simulink model "SUB_ExpIOControl"  (R2018b)
(part 5 of 6)

  out_OUT_ACAN.BSG_EXPA.OUT_12 : KIBES_Signal/KIBES_Signal  MBDS_LibraryBlock=on  DatabaseKey=932  SignalName=OUT_ACAN.BSG_EXPA.OUT_12  SymbolName=OUT_ACAN_BSG_EXPA_OUT_12_000932  DataType=boolean  Init=0  Slope=1  Bias=0  DataSize=1  fpDataType=boolean  BlockIOType=Outport  DeviceType=0
  out_OUT_ACAN.BSG_EXPA.OUT_12_TD_START : KIBES_Signal/KIBES_Signal  MBDS_LibraryBlock=on  DatabaseKey=928  SignalName=OUT_ACAN.BSG_EXPA.OUT_12_TD_START  SymbolName=OUT_ACAN_BSG_EXPA_OUT_12_TD_START_000928  DataType=boolean  Init=0  Slope=1  Bias=0  DataSize=1  fpDataType=boolean  BlockIOType=Outport  DeviceType=0
  out_OUT_ACAN.BSG_EXPA.OUT_13 : KIBES_Signal/KIBES_Signal  MBDS_LibraryBlock=on  DatabaseKey=911  SignalName=OUT_ACAN.BSG_EXPA.OUT_13  SymbolName=OUT_ACAN_BSG_EXPA_OUT_13_000911  DataType=boolean  Init=0  Slope=1  Bias=0  DataSize=1  fpDataType=boolean  BlockIOType=Outport  DeviceType=0
  out_OUT_ACAN.BSG_EXPA.OUT_14 : KIBES_Signal/KIBES_Signal  MBDS_LibraryBlock=on  DatabaseKey=964  SignalName=OUT_ACAN.BSG_EXPA.OUT_14  SymbolName=OUT_ACAN_BSG_EXPA_OUT_14_000964  DataType=boolean  Init=0  Slope=1  Bias=0  DataSize=1  fpDataType=boolean  BlockIOType=Outport  DeviceType=0
  out_OUT_ACAN.BSG_EXPA.OUT_15 : KIBES_Signal/KIBES_Signal  MBDS_LibraryBlock=on  DatabaseKey=924  SignalName=OUT_ACAN.BSG_EXPA.OUT_15  SymbolName=OUT_ACAN_BSG_EXPA_OUT_15_000924  DataType=boolean  Init=0  Slope=1  Bias=0  DataSize=1  fpDataType=boolean  BlockIOType=Outport  DeviceType=0
  out_OUT_ACAN.BSG_EXPA.OUT_16 : KIBES_Signal/KIBES_Signal  MBDS_LibraryBlock=on  DatabaseKey=921  SignalName=OUT_ACAN.BSG_EXPA.OUT_16  SymbolName=OUT_ACAN_BSG_EXPA_OUT_16_000921  DataType=boolean  Init=0  Slope=1  Bias=0  DataSize=1  fpDataType=boolean  BlockIOType=Outport  DeviceType=0
  out_OUT_ACAN.BSG_EXPA.OUT_17 : KIBES_Signal/KIBES_Signal  MBDS_LibraryBlock=on  DatabaseKey=946  SignalName=OUT_ACAN.BSG_EXPA.OUT_17  SymbolName=OUT_ACAN_BSG_EXPA_OUT_17_000946  DataType=boolean  Init=0  Slope=1  Bias=0  DataSize=1  fpDataType=boolean  BlockIOType=Outport  DeviceType=0
  out_OUT_ACAN.BSG_EXPA.OUT_18 : KIBES_Signal/KIBES_Signal  MBDS_LibraryBlock=on  DatabaseKey=943  SignalName=OUT_ACAN.BSG_EXPA.OUT_18  SymbolName=OUT_ACAN_BSG_EXPA_OUT_18_000943  DataType=boolean  Init=0  Slope=1  Bias=0  DataSize=1  fpDataType=boolean  BlockIOType=Outport  DeviceType=0
  out_OUT_ACAN.BSG_EXPA.OUT_19 : KIBES_Signal/KIBES_Signal  MBDS_LibraryBlock=on  DatabaseKey=930  SignalName=OUT_ACAN.BSG_EXPA.OUT_19  SymbolName=OUT_ACAN_BSG_EXPA_OUT_19_000930  DataType=boolean  Init=0  Slope=1  Bias=0  DataSize=1  fpDataType=boolean  BlockIOType=Outport  DeviceType=0
  out_OUT_ACAN.BSG_EXPA.OUT_20 : KIBES_Signal/KIBES_Signal  MBDS_LibraryBlock=on  DatabaseKey=949  SignalName=OUT_ACAN.BSG_EXPA.OUT_20  SymbolName=OUT_ACAN_BSG_EXPA_OUT_20_000949  DataType=boolean  Init=0  Slope=1  Bias=0  DataSize=1  fpDataType=boolean  BlockIOType=Outport  DeviceType=0
  out_OUT_ACAN.BSG_EXPA.OUT_21 : KIBES_Signal/KIBES_Signal  MBDS_LibraryBlock=on  DatabaseKey=954  SignalName=OUT_ACAN.BSG_EXPA.OUT_21  SymbolName=OUT_ACAN_BSG_EXPA_OUT_21_000954  DataType=boolean  Init=0  Slope=1  Bias=0  DataSize=1  fpDataType=boolean  BlockIOType=Outport  DeviceType=0
  out_OUT_ACAN.BSG_EXPA.OUT_21_TD_START : KIBES_Signal/KIBES_Signal  MBDS_LibraryBlock=on  DatabaseKey=971  SignalName=OUT_ACAN.BSG_EXPA.OUT_21_TD_START  SymbolName=OUT_ACAN_BSG_EXPA_OUT_21_TD_START_000971  DataType=boolean  Init=0  Slope=1  Bias=0  DataSize=1  fpDataType=boolean  BlockIOType=Outport  DeviceType=0
  out_OUT_ACAN.BSG_EXPA.OUT_22 : KIBES_Signal/KIBES_Signal  MBDS_LibraryBlock=on  DatabaseKey=952  SignalName=OUT_ACAN.BSG_EXPA.OUT_22  SymbolName=OUT_ACAN_BSG_EXPA_OUT_22_000952  DataType=boolean  Init=0  Slope=1  Bias=0  DataSize=1  fpDataType=boolean  BlockIOType=Outport  DeviceType=0
  out_OUT_ACAN.BSG_EXPA.OUT_23 : KIBES_Signal/KIBES_Signal  MBDS_LibraryBlock=on  DatabaseKey=970  SignalName=OUT_ACAN.BSG_EXPA.OUT_23  SymbolName=OUT_ACAN_BSG_EXPA_OUT_23_000970  DataType=boolean  Init=0  Slope=1  Bias=0  DataSize=1  fpDataType=boolean  BlockIOType=Outport  DeviceType=0
  out_OUT_ACAN.BSG_EXPA.OUT_24 : KIBES_Signal/KIBES_Signal  MBDS_LibraryBlock=on  DatabaseKey=927  SignalName=OUT_ACAN.BSG_EXPA.OUT_24  SymbolName=OUT_ACAN_BSG_EXPA_OUT_24_000927  DataType=boolean  Init=0  Slope=1  Bias=0  DataSize=1  fpDataType=boolean  BlockIOType=Outport  DeviceType=0
  out_OUT_ACAN.BSG_EXPA.OUT_25 : KIBES_Signal/KIBES_Signal  MBDS_LibraryBlock=on  DatabaseKey=953  SignalName=OUT_ACAN.BSG_EXPA.OUT_25  SymbolName=OUT_ACAN_BSG_EXPA_OUT_25_000953  DataType=boolean  Init=0  Slope=1  Bias=0  DataSize=1  fpDataType=boolean  BlockIOType=Outport  DeviceType=0
  out_OUT_ACAN.BSG_EXPA.OUT_26 : KIBES_Signal/KIBES_Signal  MBDS_LibraryBlock=on  DatabaseKey=913  SignalName=OUT_ACAN.BSG_EXPA.OUT_26  SymbolName=OUT_ACAN_BSG_EXPA_OUT_26_000913  DataType=boolean  Init=0  Slope=1  Bias=0  DataSize=1  fpDataType=boolean  BlockIOType=Outport  DeviceType=0
  out_OUT_ACAN.BSG_EXPA.OUT_27 : KIBES_Signal/KIBES_Signal  MBDS_LibraryBlock=on  DatabaseKey=919  SignalName=OUT_ACAN.BSG_EXPA.OUT_27  SymbolName=OUT_ACAN_BSG_EXPA_OUT_27_000919  DataType=boolean  Init=0  Slope=1  Bias=0  DataSize=1  fpDataType=boolean  BlockIOType=Outport  DeviceType=0
  out_OUT_ACAN.BSG_EXPA.OUT_28 : KIBES_Signal/KIBES_Signal  MBDS_LibraryBlock=on  DatabaseKey=916  SignalName=OUT_ACAN.BSG_EXPA.OUT_28  SymbolName=OUT_ACAN_BSG_EXPA_OUT_28_000916  DataType=boolean  Init=0  Slope=1  Bias=0  DataSize=1  fpDataType=boolean  BlockIOType=Outport  DeviceType=0
  out_OUT_ACAN.BSG_EXPA.OUT_29_HB : KIBES_Signal/KIBES_Signal  MBDS_LibraryBlock=on  DatabaseKey=2301  SignalName=OUT_ACAN.BSG_EXPA.OUT_29_HB  SymbolName=OUT_ACAN_BSG_EXPA_OUT_29_HB_002301  DataType=int8  Init=0  Slope=1  Bias=0  DataSize=1  fpDataType=int8  BlockIOType=Outport  DeviceType=0
  out_OUT_ACAN.BSG_EXPA.OUT_30_HB : KIBES_Signal/KIBES_Signal  MBDS_LibraryBlock=on  DatabaseKey=2303  SignalName=OUT_ACAN.BSG_EXPA.OUT_30_HB  SymbolName=OUT_ACAN_BSG_EXPA_OUT_30_HB_002303  DataType=int8  Init=0  Slope=1  Bias=0  DataSize=1  fpDataType=int8  BlockIOType=Outport  DeviceType=0
  out_OUT_ACAN.BSG_EXPA.OUT_31_HB : KIBES_Signal/KIBES_Signal  MBDS_LibraryBlock=on  DatabaseKey=2305  SignalName=OUT_ACAN.BSG_EXPA.OUT_31_HB  SymbolName=OUT_ACAN_BSG_EXPA_OUT_31_HB_002305  DataType=int8  Init=0  Slope=1  Bias=0  DataSize=1  fpDataType=int8  BlockIOType=Outport  DeviceType=0
  out_OUT_ACAN.BSG_EXPA.OUT_32_HB : KIBES_Signal/KIBES_Signal  MBDS_LibraryBlock=on  DatabaseKey=2307  SignalName=OUT_ACAN.BSG_EXPA.OUT_32_HB  SymbolName=OUT_ACAN_BSG_EXPA_OUT_32_HB_002307  DataType=int8  Init=0  Slope=1  Bias=0  DataSize=1  fpDataType=int8  BlockIOType=Outport  DeviceType=0
  out_OUT_ACAN.BSG_EXPA.OUT_33_HB : KIBES_Signal/KIBES_Signal  MBDS_LibraryBlock=on  DatabaseKey=2309  SignalName=OUT_ACAN.BSG_EXPA.OUT_33_HB  SymbolName=OUT_ACAN_BSG_EXPA_OUT_33_HB_002309  DataType=int8  Init=0  Slope=1  Bias=0  DataSize=1  fpDataType=int8  BlockIOType=Outport  DeviceType=0
  out_OUT_ACAN.BSG_EXPA.OUT_34_HB : KIBES_Signal/KIBES_Signal  MBDS_LibraryBlock=on  DatabaseKey=2311  SignalName=OUT_ACAN.BSG_EXPA.OUT_34_HB  SymbolName=OUT_ACAN_BSG_EXPA_OUT_34_HB_002311  DataType=int8  Init=0  Slope=1  Bias=0  DataSize=1  fpDataType=int8  BlockIOType=Outport  DeviceType=0
  out_OUT_ACAN.BSG_EXPA.OUT_OLD_01 : KIBES_Signal/KIBES_Signal  MBDS_LibraryBlock=on  DatabaseKey=959  SignalName=OUT_ACAN.BSG_EXPA.OUT_OLD_01  SymbolName=OUT_ACAN_BSG_EXPA_OUT_OLD_01_000959  DataType=boolean  Init=0  Slope=1  Bias=0  DataSize=1  fpDataType=boolean  BlockIOType=Outport  DeviceType=0
  out_OUT_ACAN.BSG_EXPA.OUT_OLD_02 : KIBES_Signal/KIBES_Signal  MBDS_LibraryBlock=on  DatabaseKey=937  SignalName=OUT_ACAN.BSG_EXPA.OUT_OLD_02  SymbolName=OUT_ACAN_BSG_EXPA_OUT_OLD_02_000937  DataType=boolean  Init=0  Slope=1  Bias=0  DataSize=1  fpDataType=boolean  BlockIOType=Outport  DeviceType=0
  out_OUT_ACAN.BSG_EXPA.OUT_OLD_03 : KIBES_Signal/KIBES_Signal  MBDS_LibraryBlock=on  DatabaseKey=895  SignalName=OUT_ACAN.BSG_EXPA.OUT_OLD_03  SymbolName=OUT_ACAN_BSG_EXPA_OUT_OLD_03_000895  DataType=boolean  Init=0  Slope=1  Bias=0  DataSize=1  fpDataType=boolean  BlockIOType=Outport  DeviceType=0
  out_OUT_ACAN.BSG_EXPA.OUT_OLD_04 : KIBES_Signal/KIBES_Signal  MBDS_LibraryBlock=on  DatabaseKey=896  SignalName=OUT_ACAN.BSG_EXPA.OUT_OLD_04  SymbolName=OUT_ACAN_BSG_EXPA_OUT_OLD_04_000896  DataType=boolean  Init=0  Slope=1  Bias=0  DataSize=1  fpDataType=boolean  BlockIOType=Outport  DeviceType=0
  out_OUT_FMSCAN.Rx_Ctrl.Out_Ctrl.MessageEnable : KIBES_Signal/KIBES_Signal  MBDS_LibraryBlock=on  DatabaseKey=2679  SignalName=OUT_FMSCAN.Rx_Ctrl.Out_Ctrl.MessageEnable  SymbolName=OUT_FMSCAN_Rx_Ctrl_Out_Ctrl_MessageEnable_002679  DataType=boolean  Init=0  Slope=1  Bias=0  DataSize=1  fpDataType=boolean  BlockIOType=Outport  DeviceType=0
  out_OUT_FMSCAN.Rx_Ctrl.Out_HB_Ctrl.MessageEnable : KIBES_Signal/KIBES_Signal  MBDS_LibraryBlock=on  DatabaseKey=2681  SignalName=OUT_FMSCAN.Rx_Ctrl.Out_HB_Ctrl.MessageEnable  SymbolName=OUT_FMSCAN_Rx_Ctrl_Out_HB_Ctrl_MessageEnable_002681  DataType=boolean  Init=0  Slope=1  Bias=0  DataSize=1  fpDataType=boolean  BlockIOType=Outport  DeviceType=0
  out_OUT_FMSCAN.Rx_Ctrl.Out_Mirror_HB_Ctrl.MessageEnable : KIBES_Signal/KIBES_Signal  MBDS_LibraryBlock=on  DatabaseKey=2683  SignalName=OUT_FMSCAN.Rx_Ctrl.Out_Mirror_HB_Ctrl.MessageEnable  SymbolName=OUT_FMSCAN_Rx_Ctrl_Out_Mirror_HB_Ctrl_MessageEnable_002683  DataType=boolean  Init=0  Slope=1  Bias=0  DataSize=1  fpDataType=boolean  BlockIOType=Outport  DeviceType=0
  out_OUT_FMSCAN.Tx_Out.Out_01_Sts.MessageEnable : KIBES_Signal/KIBES_Signal  MBDS_LibraryBlock=on  DatabaseKey=2542  SignalName=OUT_FMSCAN.Tx_Out.Out_01_Sts.MessageEnable  SymbolName=OUT_FMSCAN_Tx_Out_Out_01_Sts_MessageEnable_002542  DataType=boolean  Init=0  Slope=1  Bias=0  DataSize=1  fpDataType=boolean  BlockIOType=Outport  DeviceType=0
  out_OUT_FMSCAN.Tx_Out.Out_01_Sts.Out_DIAG : KIBES_Signal/KIBES_Signal  MBDS_LibraryBlock=on  DatabaseKey=2432  SignalName=OUT_FMSCAN.Tx_Out.Out_01_Sts.Out_DIAG  SymbolName=OUT_FMSCAN_Tx_Out_Out_01_Sts_Out_DIAG_002432  DataType=uint16  Init=0  Slope=1  Bias=0  DataSize=1  fpDataType=uint16  BlockIOType=Outport  DeviceType=0
  out_OUT_FMSCAN.Tx_Out.Out_01_Sts.Out_SENSE : KIBES_Signal/KIBES_Signal  MBDS_LibraryBlock=on  DatabaseKey=2433  SignalName=OUT_FMSCAN.Tx_Out.Out_01_Sts.Out_SENSE  SymbolName=OUT_FMSCAN_Tx_Out_Out_01_Sts_Out_SENSE_002433  DataType=uint16  Init=0  Slope=1  Bias=0  DataSize=1  fpDataType=uint16  BlockIOType=Outport  DeviceType=0
  out_OUT_FMSCAN.Tx_Out.Out_01_Sts.Out_STATUS : KIBES_Signal/KIBES_Signal  MBDS_LibraryBlock=on  DatabaseKey=2434  SignalName=OUT_FMSCAN.Tx_Out.Out_01_Sts.Out_STATUS  SymbolName=OUT_FMSCAN_Tx_Out_Out_01_Sts_Out_STATUS_002434  DataType=uint8  Init=0  Slope=1  Bias=0  DataSize=1  fpDataType=uint8  BlockIOType=Outport  DeviceType=0
  out_OUT_FMSCAN.Tx_Out.Out_02_Sts.MessageEnable : KIBES_Signal/KIBES_Signal  MBDS_LibraryBlock=on  DatabaseKey=2543  SignalName=OUT_FMSCAN.Tx_Out.Out_02_Sts.MessageEnable  SymbolName=OUT_FMSCAN_Tx_Out_Out_02_Sts_MessageEnable_002543  DataType=boolean  Init=0  Slope=1  Bias=0  DataSize=1  fpDataType=boolean  BlockIOType=Outport  DeviceType=0
  out_OUT_FMSCAN.Tx_Out.Out_02_Sts.Out_DIAG : KIBES_Signal/KIBES_Signal  MBDS_LibraryBlock=on  DatabaseKey=2435  SignalName=OUT_FMSCAN.Tx_Out.Out_02_Sts.Out_DIAG  SymbolName=OUT_FMSCAN_Tx_Out_Out_02_Sts_Out_DIAG_002435  DataType=uint16  Init=0  Slope=1  Bias=0  DataSize=1  fpDataType=uint16  BlockIOType=Outport  DeviceType=0
  out_OUT_FMSCAN.Tx_Out.Out_02_Sts.Out_SENSE : KIBES_Signal/KIBES_Signal  MBDS_LibraryBlock=on  DatabaseKey=2436  SignalName=OUT_FMSCAN.Tx_Out.Out_02_Sts.Out_SENSE  SymbolName=OUT_FMSCAN_Tx_Out_Out_02_Sts_Out_SENSE_002436  DataType=uint16  Init=0  Slope=1  Bias=0  DataSize=1  fpDataType=uint16  BlockIOType=Outport  DeviceType=0
  out_OUT_FMSCAN.Tx_Out.Out_02_Sts.Out_STATUS : KIBES_Signal/KIBES_Signal  MBDS_LibraryBlock=on  DatabaseKey=2437  SignalName=OUT_FMSCAN.Tx_Out.Out_02_Sts.Out_STATUS  SymbolName=OUT_FMSCAN_Tx_Out_Out_02_Sts_Out_STATUS_002437  DataType=uint8  Init=0  Slope=1  Bias=0  DataSize=1  fpDataType=uint8  BlockIOType=Outport  DeviceType=0
  out_OUT_FMSCAN.Tx_Out.Out_03_Sts.MessageEnable : KIBES_Signal/KIBES_Signal  MBDS_LibraryBlock=on  DatabaseKey=2544  SignalName=OUT_FMSCAN.Tx_Out.Out_03_Sts.MessageEnable  SymbolName=OUT_FMSCAN_Tx_Out_Out_03_Sts_MessageEnable_002544  DataType=boolean  Init=0  Slope=1  Bias=0  DataSize=1  fpDataType=boolean  BlockIOType=Outport  DeviceType=0
  out_OUT_FMSCAN.Tx_Out.Out_03_Sts.Out_DIAG : KIBES_Signal/KIBES_Signal  MBDS_LibraryBlock=on  DatabaseKey=2438  SignalName=OUT_FMSCAN.Tx_Out.Out_03_Sts.Out_DIAG  SymbolName=OUT_FMSCAN_Tx_Out_Out_03_Sts_Out_DIAG_002438  DataType=uint16  Init=0  Slope=1  Bias=0  DataSize=1  fpDataType=uint16  BlockIOType=Outport  DeviceType=0
  out_OUT_FMSCAN.Tx_Out.Out_03_Sts.Out_SENSE : KIBES_Signal/KIBES_Signal  MBDS_LibraryBlock=on  DatabaseKey=2439  SignalName=OUT_FMSCAN.Tx_Out.Out_03_Sts.Out_SENSE  SymbolName=OUT_FMSCAN_Tx_Out_Out_03_Sts_Out_SENSE_002439  DataType=uint16  Init=0  Slope=1  Bias=0  DataSize=1  fpDataType=uint16  BlockIOType=Outport  DeviceType=0
  out_OUT_FMSCAN.Tx_Out.Out_03_Sts.Out_STATUS : KIBES_Signal/KIBES_Signal  MBDS_LibraryBlock=on  DatabaseKey=2440  SignalName=OUT_FMSCAN.Tx_Out.Out_03_Sts.Out_STATUS  SymbolName=OUT_FMSCAN_Tx_Out_Out_03_Sts_Out_STATUS_002440  DataType=uint8  Init=0  Slope=1  Bias=0  DataSize=1  fpDataType=uint8  BlockIOType=Outport  DeviceType=0
  out_OUT_FMSCAN.Tx_Out.Out_04_Sts.MessageEnable : KIBES_Signal/KIBES_Signal  MBDS_LibraryBlock=on  DatabaseKey=2545  SignalName=OUT_FMSCAN.Tx_Out.Out_04_Sts.MessageEnable  SymbolName=OUT_FMSCAN_Tx_Out_Out_04_Sts_MessageEnable_002545  DataType=boolean  Init=0  Slope=1  Bias=0  DataSize=1  fpDataType=boolean  BlockIOType=Outport  DeviceType=0
  out_OUT_FMSCAN.Tx_Out.Out_04_Sts.Out_DIAG : KIBES_Signal/KIBES_Signal  MBDS_LibraryBlock=on  DatabaseKey=2441  SignalName=OUT_FMSCAN.Tx_Out.Out_04_Sts.Out_DIAG  SymbolName=OUT_FMSCAN_Tx_Out_Out_04_Sts_Out_DIAG_002441  DataType=uint16  Init=0  Slope=1  Bias=0  DataSize=1  fpDataType=uint16  BlockIOType=Outport  DeviceType=0
  out_OUT_FMSCAN.Tx_Out.Out_04_Sts.Out_SENSE : KIBES_Signal/KIBES_Signal  MBDS_LibraryBlock=on  DatabaseKey=2442  SignalName=OUT_FMSCAN.Tx_Out.Out_04_Sts.Out_SENSE  SymbolName=OUT_FMSCAN_Tx_Out_Out_04_Sts_Out_SENSE_002442  DataType=uint16  Init=0  Slope=1  Bias=0  DataSize=1  fpDataType=uint16  BlockIOType=Outport  DeviceType=0
  out_OUT_FMSCAN.Tx_Out.Out_04_Sts.Out_STATUS : KIBES_Signal/KIBES_Signal  MBDS_LibraryBlock=on  DatabaseKey=2443  SignalName=OUT_FMSCAN.Tx_Out.Out_04_Sts.Out_STATUS  SymbolName=OUT_FMSCAN_Tx_Out_Out_04_Sts_Out_STATUS_002443  DataType=uint8  Init=0  Slope=1  Bias=0  DataSize=1  fpDataType=uint8  BlockIOType=Outport  DeviceType=0
  out_OUT_FMSCAN.Tx_Out.Out_05_Sts.MessageEnable : KIBES_Signal/KIBES_Signal  MBDS_LibraryBlock=on  DatabaseKey=2546  SignalName=OUT_FMSCAN.Tx_Out.Out_05_Sts.MessageEnable  SymbolName=OUT_FMSCAN_Tx_Out_Out_05_Sts_MessageEnable_002546  DataType=boolean  Init=0  Slope=1  Bias=0  DataSize=1  fpDataType=boolean  BlockIOType=Outport  DeviceType=0
  out_OUT_FMSCAN.Tx_Out.Out_05_Sts.Out_DIAG : KIBES_Signal/KIBES_Signal  MBDS_LibraryBlock=on  DatabaseKey=2444  SignalName=OUT_FMSCAN.Tx_Out.Out_05_Sts.Out_DIAG  SymbolName=OUT_FMSCAN_Tx_Out_Out_05_Sts_Out_DIAG_002444  DataType=uint16  Init=0  Slope=1  Bias=0  DataSize=1  fpDataType=uint16  BlockIOType=Outport  DeviceType=0
  out_OUT_FMSCAN.Tx_Out.Out_05_Sts.Out_SENSE : KIBES_Signal/KIBES_Signal  MBDS_LibraryBlock=on  DatabaseKey=2445  SignalName=OUT_FMSCAN.Tx_Out.Out_05_Sts.Out_SENSE  SymbolName=OUT_FMSCAN_Tx_Out_Out_05_Sts_Out_SENSE_002445  DataType=uint16  Init=0  Slope=1  Bias=0  DataSize=1  fpDataType=uint16  BlockIOType=Outport  DeviceType=0
  out_OUT_FMSCAN.Tx_Out.Out_05_Sts.Out_STATUS : KIBES_Signal/KIBES_Signal  MBDS_LibraryBlock=on  DatabaseKey=2446  SignalName=OUT_FMSCAN.Tx_Out.Out_05_Sts.Out_STATUS  SymbolName=OUT_FMSCAN_Tx_Out_Out_05_Sts_Out_STATUS_002446  DataType=uint8  Init=0  Slope=1  Bias=0  DataSize=1  fpDataType=uint8  BlockIOType=Outport  DeviceType=0
  out_OUT_FMSCAN.Tx_Out.Out_06_Sts.MessageEnable : KIBES_Signal/KIBES_Signal  MBDS_LibraryBlock=on  DatabaseKey=2547  SignalName=OUT_FMSCAN.Tx_Out.Out_06_Sts.MessageEnable  SymbolName=OUT_FMSCAN_Tx_Out_Out_06_Sts_MessageEnable_002547  DataType=boolean  Init=0  Slope=1  Bias=0  DataSize=1  fpDataType=boolean  BlockIOType=Outport  DeviceType=0
  out_OUT_FMSCAN.Tx_Out.Out_06_Sts.Out_DIAG : KIBES_Signal/KIBES_Signal  MBDS_LibraryBlock=on  DatabaseKey=2447  SignalName=OUT_FMSCAN.Tx_Out.Out_06_Sts.Out_DIAG  SymbolName=OUT_FMSCAN_Tx_Out_Out_06_Sts_Out_DIAG_002447  DataType=uint16  Init=0  Slope=1  Bias=0  DataSize=1  fpDataType=uint16  BlockIOType=Outport  DeviceType=0
  out_OUT_FMSCAN.Tx_Out.Out_06_Sts.Out_SENSE : KIBES_Signal/KIBES_Signal  MBDS_LibraryBlock=on  DatabaseKey=2448  SignalName=OUT_FMSCAN.Tx_Out.Out_06_Sts.Out_SENSE  SymbolName=OUT_FMSCAN_Tx_Out_Out_06_Sts_Out_SENSE_002448  DataType=uint16  Init=0  Slope=1  Bias=0  DataSize=1  fpDataType=uint16  BlockIOType=Outport  DeviceType=0
  out_OUT_FMSCAN.Tx_Out.Out_06_Sts.Out_STATUS : KIBES_Signal/KIBES_Signal  MBDS_LibraryBlock=on  DatabaseKey=2449  SignalName=OUT_FMSCAN.Tx_Out.Out_06_Sts.Out_STATUS  SymbolName=OUT_FMSCAN_Tx_Out_Out_06_Sts_Out_STATUS_002449  DataType=uint8  Init=0  Slope=1  Bias=0  DataSize=1  fpDataType=uint8  BlockIOType=Outport  DeviceType=0
  out_OUT_FMSCAN.Tx_Out.Out_07_Sts.MessageEnable : KIBES_Signal/KIBES_Signal  MBDS_LibraryBlock=on  DatabaseKey=2548  SignalName=OUT_FMSCAN.Tx_Out.Out_07_Sts.MessageEnable  SymbolName=OUT_FMSCAN_Tx_Out_Out_07_Sts_MessageEnable_002548  DataType=boolean  Init=0  Slope=1  Bias=0  DataSize=1  fpDataType=boolean  BlockIOType=Outport  DeviceType=0
  out_OUT_FMSCAN.Tx_Out.Out_07_Sts.Out_DIAG : KIBES_Signal/KIBES_Signal  MBDS_LibraryBlock=on  DatabaseKey=2450  SignalName=OUT_FMSCAN.Tx_Out.Out_07_Sts.Out_DIAG  SymbolName=OUT_FMSCAN_Tx_Out_Out_07_Sts_Out_DIAG_002450  DataType=uint16  Init=0  Slope=1  Bias=0  DataSize=1  fpDataType=uint16  BlockIOType=Outport  DeviceType=0
  out_OUT_FMSCAN.Tx_Out.Out_07_Sts.Out_SENSE : KIBES_Signal/KIBES_Signal  MBDS_LibraryBlock=on  DatabaseKey=2451  SignalName=OUT_FMSCAN.Tx_Out.Out_07_Sts.Out_SENSE  SymbolName=OUT_FMSCAN_Tx_Out_Out_07_Sts_Out_SENSE_002451  DataType=uint16  Init=0  Slope=1  Bias=0  DataSize=1  fpDataType=uint16  BlockIOType=Outport  DeviceType=0
  out_OUT_FMSCAN.Tx_Out.Out_07_Sts.Out_STATUS : KIBES_Signal/KIBES_Signal  MBDS_LibraryBlock=on  DatabaseKey=2452  SignalName=OUT_FMSCAN.Tx_Out.Out_07_Sts.Out_STATUS  SymbolName=OUT_FMSCAN_Tx_Out_Out_07_Sts_Out_STATUS_002452  DataType=uint8  Init=0  Slope=1  Bias=0  DataSize=1  fpDataType=uint8  BlockIOType=Outport  DeviceType=0
  out_OUT_FMSCAN.Tx_Out.Out_08_Sts.MessageEnable : KIBES_Signal/KIBES_Signal  MBDS_LibraryBlock=on  DatabaseKey=2549  SignalName=OUT_FMSCAN.Tx_Out.Out_08_Sts.MessageEnable  SymbolName=OUT_FMSCAN_Tx_Out_Out_08_Sts_MessageEnable_002549  DataType=boolean  Init=0  Slope=1  Bias=0  DataSize=1  fpDataType=boolean  BlockIOType=Outport  DeviceType=0
  out_OUT_FMSCAN.Tx_Out.Out_08_Sts.Out_DIAG : KIBES_Signal/KIBES_Signal  MBDS_LibraryBlock=on  DatabaseKey=2453  SignalName=OUT_FMSCAN.Tx_Out.Out_08_Sts.Out_DIAG  SymbolName=OUT_FMSCAN_Tx_Out_Out_08_Sts_Out_DIAG_002453  DataType=uint16  Init=0  Slope=1  Bias=0  DataSize=1  fpDataType=uint16  BlockIOType=Outport  DeviceType=0
  out_OUT_FMSCAN.Tx_Out.Out_08_Sts.Out_SENSE : KIBES_Signal/KIBES_Signal  MBDS_LibraryBlock=on  DatabaseKey=2454  SignalName=OUT_FMSCAN.Tx_Out.Out_08_Sts.Out_SENSE  SymbolName=OUT_FMSCAN_Tx_Out_Out_08_Sts_Out_SENSE_002454  DataType=uint16  Init=0  Slope=1  Bias=0  DataSize=1  fpDataType=uint16  BlockIOType=Outport  DeviceType=0
  out_OUT_FMSCAN.Tx_Out.Out_08_Sts.Out_STATUS : KIBES_Signal/KIBES_Signal  MBDS_LibraryBlock=on  DatabaseKey=2455  SignalName=OUT_FMSCAN.Tx_Out.Out_08_Sts.Out_STATUS  SymbolName=OUT_FMSCAN_Tx_Out_Out_08_Sts_Out_STATUS_002455  DataType=uint8  Init=0  Slope=1  Bias=0  DataSize=1  fpDataType=uint8  BlockIOType=Outport  DeviceType=0
  out_OUT_FMSCAN.Tx_Out.Out_09_Sts.MessageEnable : KIBES_Signal/KIBES_Signal  MBDS_LibraryBlock=on  DatabaseKey=2550  SignalName=OUT_FMSCAN.Tx_Out.Out_09_Sts.MessageEnable  SymbolName=OUT_FMSCAN_Tx_Out_Out_09_Sts_MessageEnable_002550  DataType=boolean  Init=0  Slope=1  Bias=0  DataSize=1  fpDataType=boolean  BlockIOType=Outport  DeviceType=0
  out_OUT_FMSCAN.Tx_Out.Out_09_Sts.Out_DIAG : KIBES_Signal/KIBES_Signal  MBDS_LibraryBlock=on  DatabaseKey=2456  SignalName=OUT_FMSCAN.Tx_Out.Out_09_Sts.Out_DIAG  SymbolName=OUT_FMSCAN_Tx_Out_Out_09_Sts_Out_DIAG_002456  DataType=uint16  Init=0  Slope=1  Bias=0  DataSize=1  fpDataType=uint16  BlockIOType=Outport  DeviceType=0
  out_OUT_FMSCAN.Tx_Out.Out_09_Sts.Out_SENSE : KIBES_Signal/KIBES_Signal  MBDS_LibraryBlock=on  DatabaseKey=2457  SignalName=OUT_FMSCAN.Tx_Out.Out_09_Sts.Out_SENSE  SymbolName=OUT_FMSCAN_Tx_Out_Out_09_Sts_Out_SENSE_002457  DataType=uint16  Init=0  Slope=1  Bias=0  DataSize=1  fpDataType=uint16  BlockIOType=Outport  DeviceType=0
  out_OUT_FMSCAN.Tx_Out.Out_09_Sts.Out_STATUS : KIBES_Signal/KIBES_Signal  MBDS_LibraryBlock=on  DatabaseKey=2458  SignalName=OUT_FMSCAN.Tx_Out.Out_09_Sts.Out_STATUS  SymbolName=OUT_FMSCAN_Tx_Out_Out_09_Sts_Out_STATUS_002458  DataType=uint8  Init=0  Slope=1  Bias=0  DataSize=1  fpDataType=uint8  BlockIOType=Outport  DeviceType=0
  out_OUT_FMSCAN.Tx_Out.Out_10_Sts.MessageEnable : KIBES_Signal/KIBES_Signal  MBDS_LibraryBlock=on  DatabaseKey=2551  SignalName=OUT_FMSCAN.Tx_Out.Out_10_Sts.MessageEnable  SymbolName=OUT_FMSCAN_Tx_Out_Out_10_Sts_MessageEnable_002551  DataType=boolean  Init=0  Slope=1  Bias=0  DataSize=1  fpDataType=boolean  BlockIOType=Outport  DeviceType=0
  out_OUT_FMSCAN.Tx_Out.Out_10_Sts.Out_DIAG : KIBES_Signal/KIBES_Signal  MBDS_LibraryBlock=on  DatabaseKey=2459  SignalName=OUT_FMSCAN.Tx_Out.Out_10_Sts.Out_DIAG  SymbolName=OUT_FMSCAN_Tx_Out_Out_10_Sts_Out_DIAG_002459  DataType=uint16  Init=0  Slope=1  Bias=0  DataSize=1  fpDataType=uint16  BlockIOType=Outport  DeviceType=0
  out_OUT_FMSCAN.Tx_Out.Out_10_Sts.Out_SENSE : KIBES_Signal/KIBES_Signal  MBDS_LibraryBlock=on  DatabaseKey=2460  SignalName=OUT_FMSCAN.Tx_Out.Out_10_Sts.Out_SENSE  SymbolName=OUT_FMSCAN_Tx_Out_Out_10_Sts_Out_SENSE_002460  DataType=uint16  Init=0  Slope=1  Bias=0  DataSize=1  fpDataType=uint16  BlockIOType=Outport  DeviceType=0
  out_OUT_FMSCAN.Tx_Out.Out_10_Sts.Out_STATUS : KIBES_Signal/KIBES_Signal  MBDS_LibraryBlock=on  DatabaseKey=2461  SignalName=OUT_FMSCAN.Tx_Out.Out_10_Sts.Out_STATUS  SymbolName=OUT_FMSCAN_Tx_Out_Out_10_Sts_Out_STATUS_002461  DataType=uint8  Init=0  Slope=1  Bias=0  DataSize=1  fpDataType=uint8  BlockIOType=Outport  DeviceType=0
  out_OUT_FMSCAN.Tx_Out.Out_11_Sts.MessageEnable : KIBES_Signal/KIBES_Signal  MBDS_LibraryBlock=on  DatabaseKey=2552  SignalName=OUT_FMSCAN.Tx_Out.Out_11_Sts.MessageEnable  SymbolName=OUT_FMSCAN_Tx_Out_Out_11_Sts_MessageEnable_002552  DataType=boolean  Init=0  Slope=1  Bias=0  DataSize=1  fpDataType=boolean  BlockIOType=Outport  DeviceType=0
  out_OUT_FMSCAN.Tx_Out.Out_11_Sts.Out_DIAG : KIBES_Signal/KIBES_Signal  MBDS_LibraryBlock=on  DatabaseKey=2462  SignalName=OUT_FMSCAN.Tx_Out.Out_11_Sts.Out_DIAG  SymbolName=OUT_FMSCAN_Tx_Out_Out_11_Sts_Out_DIAG_002462  DataType=uint16  Init=0  Slope=1  Bias=0  DataSize=1  fpDataType=uint16  BlockIOType=Outport  DeviceType=0
  out_OUT_FMSCAN.Tx_Out.Out_11_Sts.Out_SENSE : KIBES_Signal/KIBES_Signal  MBDS_LibraryBlock=on  DatabaseKey=2463  SignalName=OUT_FMSCAN.Tx_Out.Out_11_Sts.Out_SENSE  SymbolName=OUT_FMSCAN_Tx_Out_Out_11_Sts_Out_SENSE_002463  DataType=uint16  Init=0  Slope=1  Bias=0  DataSize=1  fpDataType=uint16  BlockIOType=Outport  DeviceType=0
  out_OUT_FMSCAN.Tx_Out.Out_11_Sts.Out_STATUS : KIBES_Signal/KIBES_Signal  MBDS_LibraryBlock=on  DatabaseKey=2464  SignalName=OUT_FMSCAN.Tx_Out.Out_11_Sts.Out_STATUS  SymbolName=OUT_FMSCAN_Tx_Out_Out_11_Sts_Out_STATUS_002464  DataType=uint8  Init=0  Slope=1  Bias=0  DataSize=1  fpDataType=uint8  BlockIOType=Outport  DeviceType=0
  out_OUT_FMSCAN.Tx_Out.Out_12_Sts.MessageEnable : KIBES_Signal/KIBES_Signal  MBDS_LibraryBlock=on  DatabaseKey=2554  SignalName=OUT_FMSCAN.Tx_Out.Out_12_Sts.MessageEnable  SymbolName=OUT_FMSCAN_Tx_Out_Out_12_Sts_MessageEnable_002554  DataType=boolean  Init=0  Slope=1  Bias=0  DataSize=1  fpDataType=boolean  BlockIOType=Outport  DeviceType=0
  out_OUT_FMSCAN.Tx_Out.Out_12_Sts.Out_DIAG : KIBES_Signal/KIBES_Signal  MBDS_LibraryBlock=on  DatabaseKey=2465  SignalName=OUT_FMSCAN.Tx_Out.Out_12_Sts.Out_DIAG  SymbolName=OUT_FMSCAN_Tx_Out_Out_12_Sts_Out_DIAG_002465  DataType=uint16  Init=0  Slope=1  Bias=0  DataSize=1  fpDataType=uint16  BlockIOType=Outport  DeviceType=0
  out_OUT_FMSCAN.Tx_Out.Out_12_Sts.Out_SENSE : KIBES_Signal/KIBES_Signal  MBDS_LibraryBlock=on  DatabaseKey=2466  SignalName=OUT_FMSCAN.Tx_Out.Out_12_Sts.Out_SENSE  SymbolName=OUT_FMSCAN_Tx_Out_Out_12_Sts_Out_SENSE_002466  DataType=uint16  Init=0  Slope=1  Bias=0  DataSize=1  fpDataType=uint16  BlockIOType=Outport  DeviceType=0
  out_OUT_FMSCAN.Tx_Out.Out_12_Sts.Out_STATUS : KIBES_Signal/KIBES_Signal  MBDS_LibraryBlock=on  DatabaseKey=2467  SignalName=OUT_FMSCAN.Tx_Out.Out_12_Sts.Out_STATUS  SymbolName=OUT_FMSCAN_Tx_Out_Out_12_Sts_Out_STATUS_002467  DataType=uint8  Init=0  Slope=1  Bias=0  DataSize=1  fpDataType=uint8  BlockIOType=Outport  DeviceType=0
  out_OUT_FMSCAN.Tx_Out.Out_12_Sts.Out_TD : KIBES_Signal/KIBES_Signal  MBDS_LibraryBlock=on  DatabaseKey=2468  SignalName=OUT_FMSCAN.Tx_Out.Out_12_Sts.Out_TD  SymbolName=OUT_FMSCAN_Tx_Out_Out_12_Sts_Out_TD_002468  DataType=boolean  Init=0  Slope=1  Bias=0  DataSize=1  fpDataType=boolean  BlockIOType=Outport  DeviceType=0
  out_OUT_FMSCAN.Tx_Out.Out_12_Sts.Out_TD_DIAG : KIBES_Signal/KIBES_Signal  MBDS_LibraryBlock=on  DatabaseKey=2469  SignalName=OUT_FMSCAN.Tx_Out.Out_12_Sts.Out_TD_DIAG  SymbolName=OUT_FMSCAN_Tx_Out_Out_12_Sts_Out_TD_DIAG_002469  DataType=uint16  Init=0  Slope=1  Bias=0  DataSize=1  fpDataType=uint16  BlockIOType=Outport  DeviceType=0
  out_OUT_FMSCAN.Tx_Out.Out_12_TD_Sts.MessageEnable : KIBES_Signal/KIBES_Signal  MBDS_LibraryBlock=on  DatabaseKey=2555  SignalName=OUT_FMSCAN.Tx_Out.Out_12_TD_Sts.MessageEnable  SymbolName=OUT_FMSCAN_Tx_Out_Out_12_TD_Sts_MessageEnable_002555  DataType=boolean  Init=0  Slope=1  Bias=0  DataSize=1  fpDataType=boolean  BlockIOType=Outport  DeviceType=0
  out_OUT_FMSCAN.Tx_Out.Out_12_TD_Sts.Out_SENSE_PULSE : KIBES_Signal/KIBES_Signal  MBDS_LibraryBlock=on  DatabaseKey=2470  SignalName=OUT_FMSCAN.Tx_Out.Out_12_TD_Sts.Out_SENSE_PULSE  SymbolName=OUT_FMSCAN_Tx_Out_Out_12_TD_Sts_Out_SENSE_PULSE_002470  DataType=uint16  Init=0  Slope=1  Bias=0  DataSize=1  fpDataType=uint16  BlockIOType=Outport  DeviceType=0
  out_OUT_FMSCAN.Tx_Out.Out_12_TD_Sts.Out_SENSE_PULSE_DIAG : KIBES_Signal/KIBES_Signal  MBDS_LibraryBlock=on  DatabaseKey=2471  SignalName=OUT_FMSCAN.Tx_Out.Out_12_TD_Sts.Out_SENSE_PULSE_DIAG  SymbolName=OUT_FMSCAN_Tx_Out_Out_12_TD_Sts_Out_SENSE_PULSE_DIAG_002471  DataType=uint16  Init=0  Slope=1  Bias=0  DataSize=1  fpDataType=uint16  BlockIOType=Outport  DeviceType=0
  out_OUT_FMSCAN.Tx_Out.Out_13_Sts.MessageEnable : KIBES_Signal/KIBES_Signal  MBDS_LibraryBlock=on  DatabaseKey=2556  SignalName=OUT_FMSCAN.Tx_Out.Out_13_Sts.MessageEnable  SymbolName=OUT_FMSCAN_Tx_Out_Out_13_Sts_MessageEnable_002556  DataType=boolean  Init=0  Slope=1  Bias=0  DataSize=1  fpDataType=boolean  BlockIOType=Outport  DeviceType=0
  out_OUT_FMSCAN.Tx_Out.Out_13_Sts.Out_DIAG : KIBES_Signal/KIBES_Signal  MBDS_LibraryBlock=on  DatabaseKey=2472  SignalName=OUT_FMSCAN.Tx_Out.Out_13_Sts.Out_DIAG  SymbolName=OUT_FMSCAN_Tx_Out_Out_13_Sts_Out_DIAG_002472  DataType=uint16  Init=0  Slope=1  Bias=0  DataSize=1  fpDataType=uint16  BlockIOType=Outport  DeviceType=0
  out_OUT_FMSCAN.Tx_Out.Out_13_Sts.Out_SENSE : KIBES_Signal/KIBES_Signal  MBDS_LibraryBlock=on  DatabaseKey=2473  SignalName=OUT_FMSCAN.Tx_Out.Out_13_Sts.Out_SENSE  SymbolName=OUT_FMSCAN_Tx_Out_Out_13_Sts_Out_SENSE_002473  DataType=uint16  Init=0  Slope=1  Bias=0  DataSize=1  fpDataType=uint16  BlockIOType=Outport  DeviceType=0
  out_OUT_FMSCAN.Tx_Out.Out_13_Sts.Out_STATUS : KIBES_Signal/KIBES_Signal  MBDS_LibraryBlock=on  DatabaseKey=2474  SignalName=OUT_FMSCAN.Tx_Out.Out_13_Sts.Out_STATUS  SymbolName=OUT_FMSCAN_Tx_Out_Out_13_Sts_Out_STATUS_002474  DataType=uint8  Init=0  Slope=1  Bias=0  DataSize=1  fpDataType=uint8  BlockIOType=Outport  DeviceType=0
  out_OUT_FMSCAN.Tx_Out.Out_14_Sts.MessageEnable : KIBES_Signal/KIBES_Signal  MBDS_LibraryBlock=on  DatabaseKey=2557  SignalName=OUT_FMSCAN.Tx_Out.Out_14_Sts.MessageEnable  SymbolName=OUT_FMSCAN_Tx_Out_Out_14_Sts_MessageEnable_002557  DataType=boolean  Init=0  Slope=1  Bias=0  DataSize=1  fpDataType=boolean  BlockIOType=Outport  DeviceType=0
  out_OUT_FMSCAN.Tx_Out.Out_14_Sts.Out_DIAG : KIBES_Signal/KIBES_Signal  MBDS_LibraryBlock=on  DatabaseKey=2475  SignalName=OUT_FMSCAN.Tx_Out.Out_14_Sts.Out_DIAG  SymbolName=OUT_FMSCAN_Tx_Out_Out_14_Sts_Out_DIAG_002475  DataType=uint16  Init=0  Slope=1  Bias=0  DataSize=1  fpDataType=uint16  BlockIOType=Outport  DeviceType=0
  out_OUT_FMSCAN.Tx_Out.Out_14_Sts.Out_SENSE : KIBES_Signal/KIBES_Signal  MBDS_LibraryBlock=on  DatabaseKey=2476  SignalName=OUT_FMSCAN.Tx_Out.Out_14_Sts.Out_SENSE  SymbolName=OUT_FMSCAN_Tx_Out_Out_14_Sts_Out_SENSE_002476  DataType=uint16  Init=0  Slope=1  Bias=0  DataSize=1  fpDataType=uint16  BlockIOType=Outport  DeviceType=0
  out_OUT_FMSCAN.Tx_Out.Out_14_Sts.Out_STATUS : KIBES_Signal/KIBES_Signal  MBDS_LibraryBlock=on  DatabaseKey=2477  SignalName=OUT_FMSCAN.Tx_Out.Out_14_Sts.Out_STATUS  SymbolName=OUT_FMSCAN_Tx_Out_Out_14_Sts_Out_STATUS_002477  DataType=uint8  Init=0  Slope=1  Bias=0  DataSize=1  fpDataType=uint8  BlockIOType=Outport  DeviceType=0
  out_OUT_FMSCAN.Tx_Out.Out_15_Sts.MessageEnable : KIBES_Signal/KIBES_Signal  MBDS_LibraryBlock=on  DatabaseKey=2558  SignalName=OUT_FMSCAN.Tx_Out.Out_15_Sts.MessageEnable  SymbolName=OUT_FMSCAN_Tx_Out_Out_15_Sts_MessageEnable_002558  DataType=boolean  Init=0  Slope=1  Bias=0  DataSize=1  fpDataType=boolean  BlockIOType=Outport  DeviceType=0
  out_OUT_FMSCAN.Tx_Out.Out_15_Sts.Out_DIAG : KIBES_Signal/KIBES_Signal  MBDS_LibraryBlock=on  DatabaseKey=2478  SignalName=OUT_FMSCAN.Tx_Out.Out_15_Sts.Out_DIAG  SymbolName=OUT_FMSCAN_Tx_Out_Out_15_Sts_Out_DIAG_002478  DataType=uint16  Init=0  Slope=1  Bias=0  DataSize=1  fpDataType=uint16  BlockIOType=Outport  DeviceType=0
  out_OUT_FMSCAN.Tx_Out.Out_15_Sts.Out_SENSE : KIBES_Signal/KIBES_Signal  MBDS_LibraryBlock=on  DatabaseKey=2479  SignalName=OUT_FMSCAN.Tx_Out.Out_15_Sts.Out_SENSE  SymbolName=OUT_FMSCAN_Tx_Out_Out_15_Sts_Out_SENSE_002479  DataType=uint16  Init=0  Slope=1  Bias=0  DataSize=1  fpDataType=uint16  BlockIOType=Outport  DeviceType=0
  out_OUT_FMSCAN.Tx_Out.Out_15_Sts.Out_STATUS : KIBES_Signal/KIBES_Signal  MBDS_LibraryBlock=on  DatabaseKey=2480  SignalName=OUT_FMSCAN.Tx_Out.Out_15_Sts.Out_STATUS  SymbolName=OUT_FMSCAN_Tx_Out_Out_15_Sts_Out_STATUS_002480  DataType=uint8  Init=0  Slope=1  Bias=0  DataSize=1  fpDataType=uint8  BlockIOType=Outport  DeviceType=0
  out_OUT_FMSCAN.Tx_Out.Out_16_Sts.MessageEnable : KIBES_Signal/KIBES_Signal  MBDS_LibraryBlock=on  DatabaseKey=2559  SignalName=OUT_FMSCAN.Tx_Out.Out_16_Sts.MessageEnable  SymbolName=OUT_FMSCAN_Tx_Out_Out_16_Sts_MessageEnable_002559  DataType=boolean  Init=0  Slope=1  Bias=0  DataSize=1  fpDataType=boolean  BlockIOType=Outport  DeviceType=0
  out_OUT_FMSCAN.Tx_Out.Out_16_Sts.Out_DIAG : KIBES_Signal/KIBES_Signal  MBDS_LibraryBlock=on  DatabaseKey=2481  SignalName=OUT_FMSCAN.Tx_Out.Out_16_Sts.Out_DIAG  SymbolName=OUT_FMSCAN_Tx_Out_Out_16_Sts_Out_DIAG_002481  DataType=uint16  Init=0  Slope=1  Bias=0  DataSize=1  fpDataType=uint16  BlockIOType=Outport  DeviceType=0
  out_OUT_FMSCAN.Tx_Out.Out_16_Sts.Out_SENSE : KIBES_Signal/KIBES_Signal  MBDS_LibraryBlock=on  DatabaseKey=2482  SignalName=OUT_FMSCAN.Tx_Out.Out_16_Sts.Out_SENSE  SymbolName=OUT_FMSCAN_Tx_Out_Out_16_Sts_Out_SENSE_002482  DataType=uint16  Init=0  Slope=1  Bias=0  DataSize=1  fpDataType=uint16  BlockIOType=Outport  DeviceType=0
  out_OUT_FMSCAN.Tx_Out.Out_16_Sts.Out_STATUS : KIBES_Signal/KIBES_Signal  MBDS_LibraryBlock=on  DatabaseKey=2483  SignalName=OUT_FMSCAN.Tx_Out.Out_16_Sts.Out_STATUS  SymbolName=OUT_FMSCAN_Tx_Out_Out_16_Sts_Out_STATUS_002483  DataType=uint8  Init=0  Slope=1  Bias=0  DataSize=1  fpDataType=uint8  BlockIOType=Outport  DeviceType=0
  out_OUT_FMSCAN.Tx_Out.Out_17_Sts.MessageEnable : KIBES_Signal/KIBES_Signal  MBDS_LibraryBlock=on  DatabaseKey=2560  SignalName=OUT_FMSCAN.Tx_Out.Out_17_Sts.MessageEnable  SymbolName=OUT_FMSCAN_Tx_Out_Out_17_Sts_MessageEnable_002560  DataType=boolean  Init=0  Slope=1  Bias=0  DataSize=1  fpDataType=boolean  BlockIOType=Outport  DeviceType=0
  out_OUT_FMSCAN.Tx_Out.Out_17_Sts.Out_DIAG : KIBES_Signal/KIBES_Signal  MBDS_LibraryBlock=on  DatabaseKey=2484  SignalName=OUT_FMSCAN.Tx_Out.Out_17_Sts.Out_DIAG  SymbolName=OUT_FMSCAN_Tx_Out_Out_17_Sts_Out_DIAG_002484  DataType=uint16  Init=0  Slope=1  Bias=0  DataSize=1  fpDataType=uint16  BlockIOType=Outport  DeviceType=0
  out_OUT_FMSCAN.Tx_Out.Out_17_Sts.Out_SENSE : KIBES_Signal/KIBES_Signal  MBDS_LibraryBlock=on  DatabaseKey=2485  SignalName=OUT_FMSCAN.Tx_Out.Out_17_Sts.Out_SENSE  SymbolName=OUT_FMSCAN_Tx_Out_Out_17_Sts_Out_SENSE_002485  DataType=uint16  Init=0  Slope=1  Bias=0  DataSize=1  fpDataType=uint16  BlockIOType=Outport  DeviceType=0
  out_OUT_FMSCAN.Tx_Out.Out_17_Sts.Out_STATUS : KIBES_Signal/KIBES_Signal  MBDS_LibraryBlock=on  DatabaseKey=2486  SignalName=OUT_FMSCAN.Tx_Out.Out_17_Sts.Out_STATUS  SymbolName=OUT_FMSCAN_Tx_Out_Out_17_Sts_Out_STATUS_002486  DataType=uint8  Init=0  Slope=1  Bias=0  DataSize=1  fpDataType=uint8  BlockIOType=Outport  DeviceType=0
  out_OUT_FMSCAN.Tx_Out.Out_18_Sts.MessageEnable : KIBES_Signal/KIBES_Signal  MBDS_LibraryBlock=on  DatabaseKey=2561  SignalName=OUT_FMSCAN.Tx_Out.Out_18_Sts.MessageEnable  SymbolName=OUT_FMSCAN_Tx_Out_Out_18_Sts_MessageEnable_002561  DataType=boolean  Init=0  Slope=1  Bias=0  DataSize=1  fpDataType=boolean  BlockIOType=Outport  DeviceType=0
  out_OUT_FMSCAN.Tx_Out.Out_18_Sts.Out_DIAG : KIBES_Signal/KIBES_Signal  MBDS_LibraryBlock=on  DatabaseKey=2487  SignalName=OUT_FMSCAN.Tx_Out.Out_18_Sts.Out_DIAG  SymbolName=OUT_FMSCAN_Tx_Out_Out_18_Sts_Out_DIAG_002487  DataType=uint16  Init=0  Slope=1  Bias=0  DataSize=1  fpDataType=uint16  BlockIOType=Outport  DeviceType=0
  out_OUT_FMSCAN.Tx_Out.Out_18_Sts.Out_SENSE : KIBES_Signal/KIBES_Signal  MBDS_LibraryBlock=on  DatabaseKey=2488  SignalName=OUT_FMSCAN.Tx_Out.Out_18_Sts.Out_SENSE  SymbolName=OUT_FMSCAN_Tx_Out_Out_18_Sts_Out_SENSE_002488  DataType=uint16  Init=0  Slope=1  Bias=0  DataSize=1  fpDataType=uint16  BlockIOType=Outport  DeviceType=0
  out_OUT_FMSCAN.Tx_Out.Out_18_Sts.Out_STATUS : KIBES_Signal/KIBES_Signal  MBDS_LibraryBlock=on  DatabaseKey=2489  SignalName=OUT_FMSCAN.Tx_Out.Out_18_Sts.Out_STATUS  SymbolName=OUT_FMSCAN_Tx_Out_Out_18_Sts_Out_STATUS_002489  DataType=uint8  Init=0  Slope=1  Bias=0  DataSize=1  fpDataType=uint8  BlockIOType=Outport  DeviceType=0
  out_OUT_FMSCAN.Tx_Out.Out_19_Sts.MessageEnable : KIBES_Signal/KIBES_Signal  MBDS_LibraryBlock=on  DatabaseKey=2562  SignalName=OUT_FMSCAN.Tx_Out.Out_19_Sts.MessageEnable  SymbolName=OUT_FMSCAN_Tx_Out_Out_19_Sts_MessageEnable_002562  DataType=boolean  Init=0  Slope=1  Bias=0  DataSize=1  fpDataType=boolean  BlockIOType=Outport  DeviceType=0
  out_OUT_FMSCAN.Tx_Out.Out_19_Sts.Out_DIAG : KIBES_Signal/KIBES_Signal  MBDS_LibraryBlock=on  DatabaseKey=2490  SignalName=OUT_FMSCAN.Tx_Out.Out_19_Sts.Out_DIAG  SymbolName=OUT_FMSCAN_Tx_Out_Out_19_Sts_Out_DIAG_002490  DataType=uint16  Init=0  Slope=1  Bias=0  DataSize=1  fpDataType=uint16  BlockIOType=Outport  DeviceType=0
  out_OUT_FMSCAN.Tx_Out.Out_19_Sts.Out_SENSE : KIBES_Signal/KIBES_Signal  MBDS_LibraryBlock=on  DatabaseKey=2491  SignalName=OUT_FMSCAN.Tx_Out.Out_19_Sts.Out_SENSE  SymbolName=OUT_FMSCAN_Tx_Out_Out_19_Sts_Out_SENSE_002491  DataType=uint16  Init=0  Slope=1  Bias=0  DataSize=1  fpDataType=uint16  BlockIOType=Outport  DeviceType=0
  out_OUT_FMSCAN.Tx_Out.Out_19_Sts.Out_STATUS : KIBES_Signal/KIBES_Signal  MBDS_LibraryBlock=on  DatabaseKey=2492  SignalName=OUT_FMSCAN.Tx_Out.Out_19_Sts.Out_STATUS  SymbolName=OUT_FMSCAN_Tx_Out_Out_19_Sts_Out_STATUS_002492  DataType=uint8  Init=0  Slope=1  Bias=0  DataSize=1  fpDataType=uint8  BlockIOType=Outport  DeviceType=0
  out_OUT_FMSCAN.Tx_Out.Out_20_Sts.MessageEnable : KIBES_Signal/KIBES_Signal  MBDS_LibraryBlock=on  DatabaseKey=2563  SignalName=OUT_FMSCAN.Tx_Out.Out_20_Sts.MessageEnable  SymbolName=OUT_FMSCAN_Tx_Out_Out_20_Sts_MessageEnable_002563  DataType=boolean  Init=0  Slope=1  Bias=0  DataSize=1  fpDataType=boolean  BlockIOType=Outport  DeviceType=0
  out_OUT_FMSCAN.Tx_Out.Out_20_Sts.Out_DIAG : KIBES_Signal/KIBES_Signal  MBDS_LibraryBlock=on  DatabaseKey=2493  SignalName=OUT_FMSCAN.Tx_Out.Out_20_Sts.Out_DIAG  SymbolName=OUT_FMSCAN_Tx_Out_Out_20_Sts_Out_DIAG_002493  DataType=uint16  Init=0  Slope=1  Bias=0  DataSize=1  fpDataType=uint16  BlockIOType=Outport  DeviceType=0
  out_OUT_FMSCAN.Tx_Out.Out_20_Sts.Out_SENSE : KIBES_Signal/KIBES_Signal  MBDS_LibraryBlock=on  DatabaseKey=2494  SignalName=OUT_FMSCAN.Tx_Out.Out_20_Sts.Out_SENSE  SymbolName=OUT_FMSCAN_Tx_Out_Out_20_Sts_Out_SENSE_002494  DataType=uint16  Init=0  Slope=1  Bias=0  DataSize=1  fpDataType=uint16  BlockIOType=Outport  DeviceType=0
  out_OUT_FMSCAN.Tx_Out.Out_20_Sts.Out_STATUS : KIBES_Signal/KIBES_Signal  MBDS_LibraryBlock=on  DatabaseKey=2495  SignalName=OUT_FMSCAN.Tx_Out.Out_20_Sts.Out_STATUS  SymbolName=OUT_FMSCAN_Tx_Out_Out_20_Sts_Out_STATUS_002495  DataType=uint8  Init=0  Slope=1  Bias=0  DataSize=1  fpDataType=uint8  BlockIOType=Outport  DeviceType=0
  out_OUT_FMSCAN.Tx_Out.Out_21_Sts.MessageEnable : KIBES_Signal/KIBES_Signal  MBDS_LibraryBlock=on  DatabaseKey=2684  SignalName=OUT_FMSCAN.Tx_Out.Out_21_Sts.MessageEnable  SymbolName=OUT_FMSCAN_Tx_Out_Out_21_Sts_MessageEnable_002684  DataType=boolean  Init=0  Slope=1  Bias=0  DataSize=1  fpDataType=boolean  BlockIOType=Outport  DeviceType=0
  out_OUT_FMSCAN.Tx_Out.Out_21_Sts.Out_DIAG : KIBES_Signal/KIBES_Signal  MBDS_LibraryBlock=on  DatabaseKey=2496  SignalName=OUT_FMSCAN.Tx_Out.Out_21_Sts.Out_DIAG  SymbolName=OUT_FMSCAN_Tx_Out_Out_21_Sts_Out_DIAG_002496  DataType=uint16  Init=0  Slope=1  Bias=0  DataSize=1  fpDataType=uint16  BlockIOType=Outport  DeviceType=0
  out_OUT_FMSCAN.Tx_Out.Out_21_Sts.Out_SENSE : KIBES_Signal/KIBES_Signal  MBDS_LibraryBlock=on  DatabaseKey=2497  SignalName=OUT_FMSCAN.Tx_Out.Out_21_Sts.Out_SENSE  SymbolName=OUT_FMSCAN_Tx_Out_Out_21_Sts_Out_SENSE_002497  DataType=uint16  Init=0  Slope=1  Bias=0  DataSize=1  fpDataType=uint16  BlockIOType=Outport  DeviceType=0
  out_OUT_FMSCAN.Tx_Out.Out_21_Sts.Out_STATUS : KIBES_Signal/KIBES_Signal  MBDS_LibraryBlock=on  DatabaseKey=2498  SignalName=OUT_FMSCAN.Tx_Out.Out_21_Sts.Out_STATUS  SymbolName=OUT_FMSCAN_Tx_Out_Out_21_Sts_Out_STATUS_002498  DataType=uint8  Init=0  Slope=1  Bias=0  DataSize=1  fpDataType=uint8  BlockIOType=Outport  DeviceType=0
  out_OUT_FMSCAN.Tx_Out.Out_21_Sts.Out_TD : KIBES_Signal/KIBES_Signal  MBDS_LibraryBlock=on  DatabaseKey=2499  SignalName=OUT_FMSCAN.Tx_Out.Out_21_Sts.Out_TD  SymbolName=OUT_FMSCAN_Tx_Out_Out_21_Sts_Out_TD_002499  DataType=boolean  Init=0  Slope=1  Bias=0  DataSize=1  fpDataType=boolean  BlockIOType=Outport  DeviceType=0
  out_OUT_FMSCAN.Tx_Out.Out_21_Sts.Out_TD_DIAG : KIBES_Signal/KIBES_Signal  MBDS_LibraryBlock=on  DatabaseKey=2500  SignalName=OUT_FMSCAN.Tx_Out.Out_21_Sts.Out_TD_DIAG  SymbolName=OUT_FMSCAN_Tx_Out_Out_21_Sts_Out_TD_DIAG_002500  DataType=uint16  Init=0  Slope=1  Bias=0  DataSize=1  fpDataType=uint16  BlockIOType=Outport  DeviceType=0
  out_OUT_FMSCAN.Tx_Out.Out_21_TD_Sts.MessageEnable : KIBES_Signal/KIBES_Signal  MBDS_LibraryBlock=on  DatabaseKey=2565  SignalName=OUT_FMSCAN.Tx_Out.Out_21_TD_Sts.MessageEnable  SymbolName=OUT_FMSCAN_Tx_Out_Out_21_TD_Sts_MessageEnable_002565  DataType=boolean  Init=0  Slope=1  Bias=0  DataSize=1  fpDataType=boolean  BlockIOType=Outport  DeviceType=0
  out_OUT_FMSCAN.Tx_Out.Out_21_TD_Sts.Out_SENSE_PULSE : KIBES_Signal/KIBES_Signal  MBDS_LibraryBlock=on  DatabaseKey=2501  SignalName=OUT_FMSCAN.Tx_Out.Out_21_TD_Sts.Out_SENSE_PULSE  SymbolName=OUT_FMSCAN_Tx_Out_Out_21_TD_Sts_Out_SENSE_PULSE_002501  DataType=uint16  Init=0  Slope=1  Bias=0  DataSize=1  fpDataType=uint16  BlockIOType=Outport  DeviceType=0
  out_OUT_FMSCAN.Tx_Out.Out_21_TD_Sts.Out_SENSE_PULSE_DIAG : KIBES_Signal/KIBES_Signal  MBDS_LibraryBlock=on  DatabaseKey=2502  SignalName=OUT_FMSCAN.Tx_Out.Out_21_TD_Sts.Out_SENSE_PULSE_DIAG  SymbolName=OUT_FMSCAN_Tx_Out_Out_21_TD_Sts_Out_SENSE_PULSE_DIAG_002502  DataType=uint16  Init=0  Slope=1  Bias=0  DataSize=1  fpDataType=uint16  BlockIOType=Outport  DeviceType=0
  out_OUT_FMSCAN.Tx_Out.Out_22_Sts.MessageEnable : KIBES_Signal/KIBES_Signal  MBDS_LibraryBlock=on  DatabaseKey=2566  SignalName=OUT_FMSCAN.Tx_Out.Out_22_Sts.MessageEnable  SymbolName=OUT_FMSCAN_Tx_Out_Out_22_Sts_MessageEnable_002566  DataType=boolean  Init=0  Slope=1  Bias=0  DataSize=1  fpDataType=boolean  BlockIOType=Outport  DeviceType=0
  out_OUT_FMSCAN.Tx_Out.Out_22_Sts.Out_DIAG : KIBES_Signal/KIBES_Signal  MBDS_LibraryBlock=on  DatabaseKey=2503  SignalName=OUT_FMSCAN.Tx_Out.Out_22_Sts.Out_DIAG  SymbolName=OUT_FMSCAN_Tx_Out_Out_22_Sts_Out_DIAG_002503  DataType=uint16  Init=0  Slope=1  Bias=0  DataSize=1  fpDataType=uint16  BlockIOType=Outport  DeviceType=0
  out_OUT_FMSCAN.Tx_Out.Out_22_Sts.Out_SENSE : KIBES_Signal/KIBES_Signal  MBDS_LibraryBlock=on  DatabaseKey=2504  SignalName=OUT_FMSCAN.Tx_Out.Out_22_Sts.Out_SENSE  SymbolName=OUT_FMSCAN_Tx_Out_Out_22_Sts_Out_SENSE_002504  DataType=uint16  Init=0  Slope=1  Bias=0  DataSize=1  fpDataType=uint16  BlockIOType=Outport  DeviceType=0
  out_OUT_FMSCAN.Tx_Out.Out_22_Sts.Out_STATUS : KIBES_Signal/KIBES_Signal  MBDS_LibraryBlock=on  DatabaseKey=2505  SignalName=OUT_FMSCAN.Tx_Out.Out_22_Sts.Out_STATUS  SymbolName=OUT_FMSCAN_Tx_Out_Out_22_Sts_Out_STATUS_002505  DataType=uint8  Init=0  Slope=1  Bias=0  DataSize=1  fpDataType=uint8  BlockIOType=Outport  DeviceType=0
  out_OUT_FMSCAN.Tx_Out.Out_23_Sts.MessageEnable : KIBES_Signal/KIBES_Signal  MBDS_LibraryBlock=on  DatabaseKey=2567  SignalName=OUT_FMSCAN.Tx_Out.Out_23_Sts.MessageEnable  SymbolName=OUT_FMSCAN_Tx_Out_Out_23_Sts_MessageEnable_002567  DataType=boolean  Init=0  Slope=1  Bias=0  DataSize=1  fpDataType=boolean  BlockIOType=Outport  DeviceType=0
  out_OUT_FMSCAN.Tx_Out.Out_23_Sts.Out_DIAG : KIBES_Signal/KIBES_Signal  MBDS_LibraryBlock=on  DatabaseKey=2506  SignalName=OUT_FMSCAN.Tx_Out.Out_23_Sts.Out_DIAG  SymbolName=OUT_FMSCAN_Tx_Out_Out_23_Sts_Out_DIAG_002506  DataType=uint16  Init=0  Slope=1  Bias=0  DataSize=1  fpDataType=uint16  BlockIOType=Outport  DeviceType=0
  out_OUT_FMSCAN.Tx_Out.Out_23_Sts.Out_SENSE : KIBES_Signal/KIBES_Signal  MBDS_LibraryBlock=on  DatabaseKey=2507  SignalName=OUT_FMSCAN.Tx_Out.Out_23_Sts.Out_SENSE  SymbolName=OUT_FMSCAN_Tx_Out_Out_23_Sts_Out_SENSE_002507  DataType=uint16  Init=0  Slope=1  Bias=0  DataSize=1  fpDataType=uint16  BlockIOType=Outport  DeviceType=0
  out_OUT_FMSCAN.Tx_Out.Out_23_Sts.Out_STATUS : KIBES_Signal/KIBES_Signal  MBDS_LibraryBlock=on  DatabaseKey=2508  SignalName=OUT_FMSCAN.Tx_Out.Out_23_Sts.Out_STATUS  SymbolName=OUT_FMSCAN_Tx_Out_Out_23_Sts_Out_STATUS_002508  DataType=uint8  Init=0  Slope=1  Bias=0  DataSize=1  fpDataType=uint8  BlockIOType=Outport  DeviceType=0
  out_OUT_FMSCAN.Tx_Out.Out_24_Sts.MessageEnable : KIBES_Signal/KIBES_Signal  MBDS_LibraryBlock=on  DatabaseKey=2568  SignalName=OUT_FMSCAN.Tx_Out.Out_24_Sts.MessageEnable  SymbolName=OUT_FMSCAN_Tx_Out_Out_24_Sts_MessageEnable_002568  DataType=boolean  Init=0  Slope=1  Bias=0  DataSize=1  fpDataType=boolean  BlockIOType=Outport  DeviceType=0
  out_OUT_FMSCAN.Tx_Out.Out_24_Sts.Out_DIAG : KIBES_Signal/KIBES_Signal  MBDS_LibraryBlock=on  DatabaseKey=2509  SignalName=OUT_FMSCAN.Tx_Out.Out_24_Sts.Out_DIAG  SymbolName=OUT_FMSCAN_Tx_Out_Out_24_Sts_Out_DIAG_002509  DataType=uint16  Init=0  Slope=1  Bias=0  DataSize=1  fpDataType=uint16  BlockIOType=Outport  DeviceType=0
  out_OUT_FMSCAN.Tx_Out.Out_24_Sts.Out_SENSE : KIBES_Signal/KIBES_Signal  MBDS_LibraryBlock=on  DatabaseKey=2510  SignalName=OUT_FMSCAN.Tx_Out.Out_24_Sts.Out_SENSE  SymbolName=OUT_FMSCAN_Tx_Out_Out_24_Sts_Out_SENSE_002510  DataType=uint16  Init=0  Slope=1  Bias=0  DataSize=1  fpDataType=uint16  BlockIOType=Outport  DeviceType=0
  out_OUT_FMSCAN.Tx_Out.Out_24_Sts.Out_STATUS : KIBES_Signal/KIBES_Signal  MBDS_LibraryBlock=on  DatabaseKey=2511  SignalName=OUT_FMSCAN.Tx_Out.Out_24_Sts.Out_STATUS  SymbolName=OUT_FMSCAN_Tx_Out_Out_24_Sts_Out_STATUS_002511  DataType=uint8  Init=0  Slope=1  Bias=0  DataSize=1  fpDataType=uint8  BlockIOType=Outport  DeviceType=0
  out_OUT_FMSCAN.Tx_Out.Out_25_Sts.MessageEnable : KIBES_Signal/KIBES_Signal  MBDS_LibraryBlock=on  DatabaseKey=2569  SignalName=OUT_FMSCAN.Tx_Out.Out_25_Sts.MessageEnable  SymbolName=OUT_FMSCAN_Tx_Out_Out_25_Sts_MessageEnable_002569  DataType=boolean  Init=0  Slope=1  Bias=0  DataSize=1  fpDataType=boolean  BlockIOType=Outport  DeviceType=0
  out_OUT_FMSCAN.Tx_Out.Out_25_Sts.Out_DIAG : KIBES_Signal/KIBES_Signal  MBDS_LibraryBlock=on  DatabaseKey=2512  SignalName=OUT_FMSCAN.Tx_Out.Out_25_Sts.Out_DIAG  SymbolName=OUT_FMSCAN_Tx_Out_Out_25_Sts_Out_DIAG_002512  DataType=uint16  Init=0  Slope=1  Bias=0  DataSize=1  fpDataType=uint16  BlockIOType=Outport  DeviceType=0
  out_OUT_FMSCAN.Tx_Out.Out_25_Sts.Out_SENSE : KIBES_Signal/KIBES_Signal  MBDS_LibraryBlock=on  DatabaseKey=2513  SignalName=OUT_FMSCAN.Tx_Out.Out_25_Sts.Out_SENSE  SymbolName=OUT_FMSCAN_Tx_Out_Out_25_Sts_Out_SENSE_002513  DataType=uint16  Init=0  Slope=1  Bias=0  DataSize=1  fpDataType=uint16  BlockIOType=Outport  DeviceType=0
  out_OUT_FMSCAN.Tx_Out.Out_25_Sts.Out_STATUS : KIBES_Signal/KIBES_Signal  MBDS_LibraryBlock=on  DatabaseKey=2514  SignalName=OUT_FMSCAN.Tx_Out.Out_25_Sts.Out_STATUS  SymbolName=OUT_FMSCAN_Tx_Out_Out_25_Sts_Out_STATUS_002514  DataType=uint8  Init=0  Slope=1  Bias=0  DataSize=1  fpDataType=uint8  BlockIOType=Outport  DeviceType=0
  out_OUT_FMSCAN.Tx_Out.Out_26_Sts.MessageEnable : KIBES_Signal/KIBES_Signal  MBDS_LibraryBlock=on  DatabaseKey=2570  SignalName=OUT_FMSCAN.Tx_Out.Out_26_Sts.MessageEnable  SymbolName=OUT_FMSCAN_Tx_Out_Out_26_Sts_MessageEnable_002570  DataType=boolean  Init=0  Slope=1  Bias=0  DataSize=1  fpDataType=boolean  BlockIOType=Outport  DeviceType=0
  out_OUT_FMSCAN.Tx_Out.Out_26_Sts.Out_DIAG : KIBES_Signal/KIBES_Signal  MBDS_LibraryBlock=on  DatabaseKey=2515  SignalName=OUT_FMSCAN.Tx_Out.Out_26_Sts.Out_DIAG  SymbolName=OUT_FMSCAN_Tx_Out_Out_26_Sts_Out_DIAG_002515  DataType=uint16  Init=0  Slope=1  Bias=0  DataSize=1  fpDataType=uint16  BlockIOType=Outport  DeviceType=0
  out_OUT_FMSCAN.Tx_Out.Out_26_Sts.Out_SENSE : KIBES_Signal/KIBES_Signal  MBDS_LibraryBlock=on  DatabaseKey=2516  SignalName=OUT_FMSCAN.Tx_Out.Out_26_Sts.Out_SENSE  SymbolName=OUT_FMSCAN_Tx_Out_Out_26_Sts_Out_SENSE_002516  DataType=uint16  Init=0  Slope=1  Bias=0  DataSize=1  fpDataType=uint16  BlockIOType=Outport  DeviceType=0
  out_OUT_FMSCAN.Tx_Out.Out_26_Sts.Out_STATUS : KIBES_Signal/KIBES_Signal  MBDS_LibraryBlock=on  DatabaseKey=2517  SignalName=OUT_FMSCAN.Tx_Out.Out_26_Sts.Out_STATUS  SymbolName=OUT_FMSCAN_Tx_Out_Out_26_Sts_Out_STATUS_002517  DataType=uint8  Init=0  Slope=1  Bias=0  DataSize=1  fpDataType=uint8  BlockIOType=Outport  DeviceType=0
  out_OUT_FMSCAN.Tx_Out.Out_27_Sts.MessageEnable : KIBES_Signal/KIBES_Signal  MBDS_LibraryBlock=on  DatabaseKey=2571  SignalName=OUT_FMSCAN.Tx_Out.Out_27_Sts.MessageEnable  SymbolName=OUT_FMSCAN_Tx_Out_Out_27_Sts_MessageEnable_002571  DataType=boolean  Init=0  Slope=1  Bias=0  DataSize=1  fpDataType=boolean  BlockIOType=Outport  DeviceType=0
  out_OUT_FMSCAN.Tx_Out.Out_27_Sts.Out_DIAG : KIBES_Signal/KIBES_Signal  MBDS_LibraryBlock=on  DatabaseKey=2518  SignalName=OUT_FMSCAN.Tx_Out.Out_27_Sts.Out_DIAG  SymbolName=OUT_FMSCAN_Tx_Out_Out_27_Sts_Out_DIAG_002518  DataType=uint16  Init=0  Slope=1  Bias=0  DataSize=1  fpDataType=uint16  BlockIOType=Outport  DeviceType=0
  out_OUT_FMSCAN.Tx_Out.Out_27_Sts.Out_SENSE : KIBES_Signal/KIBES_Signal  MBDS_LibraryBlock=on  DatabaseKey=2519  SignalName=OUT_FMSCAN.Tx_Out.Out_27_Sts.Out_SENSE  SymbolName=OUT_FMSCAN_Tx_Out_Out_27_Sts_Out_SENSE_002519  DataType=uint16  Init=0  Slope=1  Bias=0  DataSize=1  fpDataType=uint16  BlockIOType=Outport  DeviceType=0
  out_OUT_FMSCAN.Tx_Out.Out_27_Sts.Out_STATUS : KIBES_Signal/KIBES_Signal  MBDS_LibraryBlock=on  DatabaseKey=2520  SignalName=OUT_FMSCAN.Tx_Out.Out_27_Sts.Out_STATUS  SymbolName=OUT_FMSCAN_Tx_Out_Out_27_Sts_Out_STATUS_002520  DataType=uint8  Init=0  Slope=1  Bias=0  DataSize=1  fpDataType=uint8  BlockIOType=Outport  DeviceType=0
  out_OUT_FMSCAN.Tx_Out.Out_28_Sts.MessageEnable : KIBES_Signal/KIBES_Signal  MBDS_LibraryBlock=on  DatabaseKey=2572  SignalName=OUT_FMSCAN.Tx_Out.Out_28_Sts.MessageEnable  SymbolName=OUT_FMSCAN_Tx_Out_Out_28_Sts_MessageEnable_002572  DataType=boolean  Init=0  Slope=1  Bias=0  DataSize=1  fpDataType=boolean  BlockIOType=Outport  DeviceType=0
  out_OUT_FMSCAN.Tx_Out.Out_28_Sts.Out_DIAG : KIBES_Signal/KIBES_Signal  MBDS_LibraryBlock=on  DatabaseKey=2521  SignalName=OUT_FMSCAN.Tx_Out.Out_28_Sts.Out_DIAG  SymbolName=OUT_FMSCAN_Tx_Out_Out_28_Sts_Out_DIAG_002521  DataType=uint16  Init=0  Slope=1  Bias=0  DataSize=1  fpDataType=uint16  BlockIOType=Outport  DeviceType=0
  out_OUT_FMSCAN.Tx_Out.Out_28_Sts.Out_SENSE : KIBES_Signal/KIBES_Signal  MBDS_LibraryBlock=on  DatabaseKey=2522  SignalName=OUT_FMSCAN.Tx_Out.Out_28_Sts.Out_SENSE  SymbolName=OUT_FMSCAN_Tx_Out_Out_28_Sts_Out_SENSE_002522  DataType=uint16  Init=0  Slope=1  Bias=0  DataSize=1  fpDataType=uint16  BlockIOType=Outport  DeviceType=0
  out_OUT_FMSCAN.Tx_Out.Out_28_Sts.Out_STATUS : KIBES_Signal/KIBES_Signal  MBDS_LibraryBlock=on  DatabaseKey=2523  SignalName=OUT_FMSCAN.Tx_Out.Out_28_Sts.Out_STATUS  SymbolName=OUT_FMSCAN_Tx_Out_Out_28_Sts_Out_STATUS_002523  DataType=uint8  Init=0  Slope=1  Bias=0  DataSize=1  fpDataType=uint8  BlockIOType=Outport  DeviceType=0
  out_OUT_FMSCAN.Tx_Out.Out_29_Sts.MessageEnable : KIBES_Signal/KIBES_Signal  MBDS_LibraryBlock=on  DatabaseKey=2573  SignalName=OUT_FMSCAN.Tx_Out.Out_29_Sts.MessageEnable  SymbolName=OUT_FMSCAN_Tx_Out_Out_29_Sts_MessageEnable_002573  DataType=boolean  Init=0  Slope=1  Bias=0  DataSize=1  fpDataType=boolean  BlockIOType=Outport  DeviceType=0
  out_OUT_FMSCAN.Tx_Out.Out_29_Sts.Out_DIAG : KIBES_Signal/KIBES_Signal  MBDS_LibraryBlock=on  DatabaseKey=2524  SignalName=OUT_FMSCAN.Tx_Out.Out_29_Sts.Out_DIAG  SymbolName=OUT_FMSCAN_Tx_Out_Out_29_Sts_Out_DIAG_002524  DataType=uint16  Init=0  Slope=1  Bias=0  DataSize=1  fpDataType=uint16  BlockIOType=Outport  DeviceType=0
  out_OUT_FMSCAN.Tx_Out.Out_29_Sts.Out_STATUS : KIBES_Signal/KIBES_Signal  MBDS_LibraryBlock=on  DatabaseKey=2526  SignalName=OUT_FMSCAN.Tx_Out.Out_29_Sts.Out_STATUS  SymbolName=OUT_FMSCAN_Tx_Out_Out_29_Sts_Out_STATUS_002526  DataType=uint8  Init=0  Slope=1  Bias=0  DataSize=1  fpDataType=uint8  BlockIOType=Outport  DeviceType=0
  out_OUT_FMSCAN.Tx_Out.Out_30_Sts.MessageEnable : KIBES_Signal/KIBES_Signal  MBDS_LibraryBlock=on  DatabaseKey=2574  SignalName=OUT_FMSCAN.Tx_Out.Out_30_Sts.MessageEnable  SymbolName=OUT_FMSCAN_Tx_Out_Out_30_Sts_MessageEnable_002574  DataType=boolean  Init=0  Slope=1  Bias=0  DataSize=1  fpDataType=boolean  BlockIOType=Outport  DeviceType=0
  out_OUT_FMSCAN.Tx_Out.Out_30_Sts.Out_DIAG : KIBES_Signal/KIBES_Signal  MBDS_LibraryBlock=on  DatabaseKey=2527  SignalName=OUT_FMSCAN.Tx_Out.Out_30_Sts.Out_DIAG  SymbolName=OUT_FMSCAN_Tx_Out_Out_30_Sts_Out_DIAG_002527  DataType=uint16  Init=0  Slope=1  Bias=0  DataSize=1  fpDataType=uint16  BlockIOType=Outport  DeviceType=0
  out_OUT_FMSCAN.Tx_Out.Out_30_Sts.Out_STATUS : KIBES_Signal/KIBES_Signal  MBDS_LibraryBlock=on  DatabaseKey=2529  SignalName=OUT_FMSCAN.Tx_Out.Out_30_Sts.Out_STATUS  SymbolName=OUT_FMSCAN_Tx_Out_Out_30_Sts_Out_STATUS_002529  DataType=uint8  Init=0  Slope=1  Bias=0  DataSize=1  fpDataType=uint8  BlockIOType=Outport  DeviceType=0
  out_OUT_FMSCAN.Tx_Out.Out_31_Sts.MessageEnable : KIBES_Signal/KIBES_Signal  MBDS_LibraryBlock=on  DatabaseKey=2575  SignalName=OUT_FMSCAN.Tx_Out.Out_31_Sts.MessageEnable  SymbolName=OUT_FMSCAN_Tx_Out_Out_31_Sts_MessageEnable_002575  DataType=boolean  Init=0  Slope=1  Bias=0  DataSize=1  fpDataType=boolean  BlockIOType=Outport  DeviceType=0
  out_OUT_FMSCAN.Tx_Out.Out_31_Sts.Out_DIAG : KIBES_Signal/KIBES_Signal  MBDS_LibraryBlock=on  DatabaseKey=2530  SignalName=OUT_FMSCAN.Tx_Out.Out_31_Sts.Out_DIAG  SymbolName=OUT_FMSCAN_Tx_Out_Out_31_Sts_Out_DIAG_002530  DataType=uint16  Init=0  Slope=1  Bias=0  DataSize=1  fpDataType=uint16  BlockIOType=Outport  DeviceType=0
  out_OUT_FMSCAN.Tx_Out.Out_31_Sts.Out_STATUS : KIBES_Signal/KIBES_Signal  MBDS_LibraryBlock=on  DatabaseKey=2532  SignalName=OUT_FMSCAN.Tx_Out.Out_31_Sts.Out_STATUS  SymbolName=OUT_FMSCAN_Tx_Out_Out_31_Sts_Out_STATUS_002532  DataType=uint8  Init=0  Slope=1  Bias=0  DataSize=1  fpDataType=uint8  BlockIOType=Outport  DeviceType=0
  out_OUT_FMSCAN.Tx_Out.Out_32_Sts.MessageEnable : KIBES_Signal/KIBES_Signal  MBDS_LibraryBlock=on  DatabaseKey=2576  SignalName=OUT_FMSCAN.Tx_Out.Out_32_Sts.MessageEnable  SymbolName=OUT_FMSCAN_Tx_Out_Out_32_Sts_MessageEnable_002576  DataType=boolean  Init=0  Slope=1  Bias=0  DataSize=1  fpDataType=boolean  BlockIOType=Outport  DeviceType=0
  out_OUT_FMSCAN.Tx_Out.Out_32_Sts.Out_DIAG : KIBES_Signal/KIBES_Signal  MBDS_LibraryBlock=on  DatabaseKey=2533  SignalName=OUT_FMSCAN.Tx_Out.Out_32_Sts.Out_DIAG  SymbolName=OUT_FMSCAN_Tx_Out_Out_32_Sts_Out_DIAG_002533  DataType=uint16  Init=0  Slope=1  Bias=0  DataSize=1  fpDataType=uint16  BlockIOType=Outport  DeviceType=0
  out_OUT_FMSCAN.Tx_Out.Out_32_Sts.Out_STATUS : KIBES_Signal/KIBES_Signal  MBDS_LibraryBlock=on  DatabaseKey=2535  SignalName=OUT_FMSCAN.Tx_Out.Out_32_Sts.Out_STATUS  SymbolName=OUT_FMSCAN_Tx_Out_Out_32_Sts_Out_STATUS_002535  DataType=uint8  Init=0  Slope=1  Bias=0  DataSize=1  fpDataType=uint8  BlockIOType=Outport  DeviceType=0
  out_OUT_FMSCAN.Tx_Out.Out_33_Sts.MessageEnable : KIBES_Signal/KIBES_Signal  MBDS_LibraryBlock=on  DatabaseKey=2577  SignalName=OUT_FMSCAN.Tx_Out.Out_33_Sts.MessageEnable  SymbolName=OUT_FMSCAN_Tx_Out_Out_33_Sts_MessageEnable_002577  DataType=boolean  Init=0  Slope=1  Bias=0  DataSize=1  fpDataType=boolean  BlockIOType=Outport  DeviceType=0
  out_OUT_FMSCAN.Tx_Out.Out_33_Sts.Out_DIAG : KIBES_Signal/KIBES_Signal  MBDS_LibraryBlock=on  DatabaseKey=2536  SignalName=OUT_FMSCAN.Tx_Out.Out_33_Sts.Out_DIAG  SymbolName=OUT_FMSCAN_Tx_Out_Out_33_Sts_Out_DIAG_002536  DataType=uint16  Init=0  Slope=1  Bias=0  DataSize=1  fpDataType=uint16  BlockIOType=Outport  DeviceType=0
  out_OUT_FMSCAN.Tx_Out.Out_33_Sts.Out_STATUS : KIBES_Signal/KIBES_Signal  MBDS_LibraryBlock=on  DatabaseKey=2538  SignalName=OUT_FMSCAN.Tx_Out.Out_33_Sts.Out_STATUS  SymbolName=OUT_FMSCAN_Tx_Out_Out_33_Sts_Out_STATUS_002538  DataType=uint8  Init=0  Slope=1  Bias=0  DataSize=1  fpDataType=uint8  BlockIOType=Outport  DeviceType=0
  out_OUT_FMSCAN.Tx_Out.Out_34_Sts.MessageEnable : KIBES_Signal/KIBES_Signal  MBDS_LibraryBlock=on  DatabaseKey=2578  SignalName=OUT_FMSCAN.Tx_Out.Out_34_Sts.MessageEnable  SymbolName=OUT_FMSCAN_Tx_Out_Out_34_Sts_MessageEnable_002578  DataType=boolean  Init=0  Slope=1  Bias=0  DataSize=1  fpDataType=boolean  BlockIOType=Outport  DeviceType=0
  out_OUT_FMSCAN.Tx_Out.Out_34_Sts.Out_DIAG : KIBES_Signal/KIBES_Signal  MBDS_LibraryBlock=on  DatabaseKey=2539  SignalName=OUT_FMSCAN.Tx_Out.Out_34_Sts.Out_DIAG  SymbolName=OUT_FMSCAN_Tx_Out_Out_34_Sts_Out_DIAG_002539  DataType=uint16  Init=0  Slope=1  Bias=0  DataSize=1  fpDataType=uint16  BlockIOType=Outport  DeviceType=0
  out_OUT_FMSCAN.Tx_Out.Out_34_Sts.Out_STATUS : KIBES_Signal/KIBES_Signal  MBDS_LibraryBlock=on  DatabaseKey=2541  SignalName=OUT_FMSCAN.Tx_Out.Out_34_Sts.Out_STATUS  SymbolName=OUT_FMSCAN_Tx_Out_Out_34_Sts_Out_STATUS_002541  DataType=uint8  Init=0  Slope=1  Bias=0  DataSize=1  fpDataType=uint8  BlockIOType=Outport  DeviceType=0
  wires:
  in_DIAG_ACAN.BSG_EXPA.OUT_13_DIAG/1 -> out_OUT_FMSCAN.Tx_Out.Out_13_Sts.Out_DIAG/1
  in_DIAG_ACAN.BSG_EXPA.OUT_12_DIAG/1 -> out_OUT_FMSCAN.Tx_Out.Out_12_Sts.Out_DIAG/1
  in_IN_ACAN.BSG_EXPA.OUT_28_SENSE/1 -> out_OUT_FMSCAN.Tx_Out.Out_28_Sts.Out_SENSE/1
  in_DIAG_ACAN.BSG_EXPA.OUT_22_DIAG/1 -> out_OUT_FMSCAN.Tx_Out.Out_22_Sts.Out_DIAG/1
  bo_SendEnable/1 -> out_OUT_FMSCAN.Tx_Out.Out_01_Sts.MessageEnable/1, out_OUT_FMSCAN.Tx_Out.Out_02_Sts.MessageEnable/1, out_OUT_FMSCAN.Tx_Out.Out_03_Sts.MessageEnable/1, out_OUT_FMSCAN.Tx_Out.Out_04_Sts.MessageEnable/1, out_OUT_FMSCAN.Tx_Out.Out_05_Sts.MessageEnable/1, out_OUT_FMSCAN.Tx_Out.Out_06_Sts.MessageEnable/1, out_OUT_FMSCAN.Tx_Out.Out_07_Sts.MessageEnable/1, out_OUT_FMSCAN.Tx_Out.Out_08_Sts.MessageEnable/1, out_OUT_FMSCAN.Tx_Out.Out_09_Sts.MessageEnable/1, out_OUT_FMSCAN.Tx_Out.Out_10_Sts.MessageEnable/1, out_OUT_FMSCAN.Tx_Out.Out_11_Sts.MessageEnable/1, out_OUT_FMSCAN.Tx_Out.Out_12_Sts.MessageEnable/1, out_OUT_FMSCAN.Tx_Out.Out_12_TD_Sts.MessageEnable/1, out_OUT_FMSCAN.Tx_Out.Out_13_Sts.MessageEnable/1, out_OUT_FMSCAN.Tx_Out.Out_14_Sts.MessageEnable/1, out_OUT_FMSCAN.Tx_Out.Out_15_Sts.MessageEnable/1, out_OUT_FMSCAN.Tx_Out.Out_16_Sts.MessageEnable/1, out_OUT_FMSCAN.Tx_Out.Out_17_Sts.MessageEnable/1, out_OUT_FMSCAN.Tx_Out.Out_18_Sts.MessageEnable/1, out_OUT_FMSCAN.Tx_Out.Out_19_Sts.MessageEnable/1, out_OUT_FMSCAN.Tx_Out.Out_20_Sts.MessageEnable/1, out_OUT_FMSCAN.Tx_Out.Out_21_Sts.MessageEnable/1, out_OUT_FMSCAN.Tx_Out.Out_21_TD_Sts.MessageEnable/1, out_OUT_FMSCAN.Tx_Out.Out_22_Sts.MessageEnable/1, out_OUT_FMSCAN.Tx_Out.Out_23_Sts.MessageEnable/1, out_OUT_FMSCAN.Tx_Out.Out_24_Sts.MessageEnable/1, out_OUT_FMSCAN.Tx_Out.Out_25_Sts.MessageEnable/1, out_OUT_FMSCAN.Tx_Out.Out_26_Sts.MessageEnable/1, out_OUT_FMSCAN.Tx_Out.Out_27_Sts.MessageEnable/1, out_OUT_FMSCAN.Tx_Out.Out_28_Sts.MessageEnable/1, out_OUT_FMSCAN.Tx_Out.Out_29_Sts.MessageEnable/1, out_OUT_FMSCAN.Tx_Out.Out_30_Sts.MessageEnable/1, out_OUT_FMSCAN.Tx_Out.Out_31_Sts.MessageEnable/1, out_OUT_FMSCAN.Tx_Out.Out_32_Sts.MessageEnable/1, out_OUT_FMSCAN.Tx_Out.Out_34_Sts.MessageEnable/1, out_OUT_FMSCAN.Tx_Out.Out_33_Sts.MessageEnable/1
  in_IN_ACAN.BSG_EXPA.OUT_13_SENSE/1 -> out_OUT_FMSCAN.Tx_Out.Out_13_Sts.Out_SENSE/1
  in_IN_ACAN.BSG_EXPA.OUT_15_SENSE/1 -> out_OUT_FMSCAN.Tx_Out.Out_15_Sts.Out_SENSE/1
  in_IN_ACAN.BSG_EXPA.OUT_21_TD/1 -> out_OUT_FMSCAN.Tx_Out.Out_21_Sts.Out_TD/1, [boOut21TD]
  in_IN_ACAN.BSG_EXPA.OUT_14_SENSE/1 -> out_OUT_FMSCAN.Tx_Out.Out_14_Sts.Out_SENSE/1
  in_IN_ACAN.BSG_EXPA.OUT_24_SENSE/1 -> out_OUT_FMSCAN.Tx_Out.Out_24_Sts.Out_SENSE/1
  in_IN_ACAN.BSG_EXPA.OUT_27_SENSE/1 -> out_OUT_FMSCAN.Tx_Out.Out_27_Sts.Out_SENSE/1
  in_IN_ACAN.BSG_EXPA.OUT_02_HB_SENSE/1 -> out_OUT_FMSCAN.Tx_Out.Out_02_Sts.Out_SENSE/1
  in_DIAG_ACAN.BSG_EXPA.OUT_07_HB_DIAG/1 -> [Out07HBDiag], out_OUT_FMSCAN.Tx_Out.Out_07_Sts.Out_DIAG/1
  in_IN_ACAN.BSG_EXPA.OUT_16_SENSE/1 -> out_OUT_FMSCAN.Tx_Out.Out_16_Sts.Out_SENSE/1
  in_DIAG_ACAN.BSG_EXPA.OUT_18_DIAG/1 -> out_OUT_FMSCAN.Tx_Out.Out_18_Sts.Out_DIAG/1
  in_DIAG_ACAN.BSG_EXPA.OUT_16_DIAG/1 -> out_OUT_FMSCAN.Tx_Out.Out_16_Sts.Out_DIAG/1
  in_DIAG_ACAN.BSG_EXPA.OUT_04_DIAG/1 -> out_OUT_FMSCAN.Tx_Out.Out_04_Sts.Out_DIAG/1
  in_DIAG_ACAN.BSG_EXPA.OUT_17_DIAG/1 -> out_OUT_FMSCAN.Tx_Out.Out_17_Sts.Out_DIAG/1
  in_DIAG_ACAN.BSG_EXPA.OUT_15_DIAG/1 -> out_OUT_FMSCAN.Tx_Out.Out_15_Sts.Out_DIAG/1
  in_DIAG_ACAN.BSG_EXPA.OUT_27_DIAG/1 -> out_OUT_FMSCAN.Tx_Out.Out_27_Sts.Out_DIAG/1
  in_IN_ACAN.BSG_EXPA.OUT_20_SENSE/1 -> out_OUT_FMSCAN.Tx_Out.Out_20_Sts.Out_SENSE/1
  in_DIAG_ACAN.BSG_EXPA.OUT_21_TD_DIAG/1 -> out_OUT_FMSCAN.Tx_Out.Out_21_Sts.Out_TD_DIAG/1, [boOut21TDDiag]
  in_DIAG_ACAN.BSG_EXPA.OUT_26_DIAG/1 -> out_OUT_FMSCAN.Tx_Out.Out_26_Sts.Out_DIAG/1
  in_DIAG_ACAN.BSG_EXPA.OUT_20_DIAG/1 -> out_OUT_FMSCAN.Tx_Out.Out_20_Sts.Out_DIAG/1
  in_IN_ACAN.BSG_EXPA.OUT_18_SENSE/1 -> out_OUT_FMSCAN.Tx_Out.Out_18_Sts.Out_SENSE/1
  in_DIAG_ACAN.BSG_EXPA.OUT_21_DIAG/1 -> out_OUT_FMSCAN.Tx_Out.Out_21_Sts.Out_DIAG/1
  in_IN_ACAN.BSG_EXPA.OUT_17_SENSE/1 -> out_OUT_FMSCAN.Tx_Out.Out_17_Sts.Out_SENSE/1
  in_DIAG_ACAN.BSG_EXPA.OUT_12_TD_DIAG/1 -> out_OUT_FMSCAN.Tx_Out.Out_12_Sts.Out_TD_DIAG/1, [boOut12TDDiag]
  in_DIAG_ACAN.BSG_EXPA.OUT_14_DIAG/1 -> out_OUT_FMSCAN.Tx_Out.Out_14_Sts.Out_DIAG/1
  in_IN_ACAN.BSG_EXPA.OUT_11_SENSE/1 -> out_OUT_FMSCAN.Tx_Out.Out_11_Sts.Out_SENSE/1
  in_DIAG_ACAN.BSG_EXPA.OUT_23_DIAG/1 -> out_OUT_FMSCAN.Tx_Out.Out_23_Sts.Out_DIAG/1
  in_DIAG_ACAN.BSG_EXPA.OUT_10_HB_DIAG/1 -> [Out10HBDiag], out_OUT_FMSCAN.Tx_Out.Out_10_Sts.Out_DIAG/1
  in_DIAG_ACAN.BSG_EXPA.OUT_25_DIAG/1 -> out_OUT_FMSCAN.Tx_Out.Out_25_Sts.Out_DIAG/1
  in_IN_ACAN.BSG_EXPA.OUT_07_HB_SENSE/1 -> out_OUT_FMSCAN.Tx_Out.Out_07_Sts.Out_SENSE/1
  in_DIAG_ACAN.BSG_EXPA.OUT_08_HB_DIAG/1 -> [Out08HBDiag], out_OUT_FMSCAN.Tx_Out.Out_08_Sts.Out_DIAG/1
  in_IN_ACAN.BSG_EXPA.OUT_03_SENSE/1 -> out_OUT_FMSCAN.Tx_Out.Out_03_Sts.Out_SENSE/1
  in_IN_ACAN.BSG_EXPA.OUT_06_HB_SENSE/1 -> out_OUT_FMSCAN.Tx_Out.Out_06_Sts.Out_SENSE/1
  in_IN_ACAN.BSG_EXPA.OUT_25_SENSE/1 -> out_OUT_FMSCAN.Tx_Out.Out_25_Sts.Out_SENSE/1
  in_IN_ACAN.BSG_EXPA.OUT_05_HB_SENSE/1 -> out_OUT_FMSCAN.Tx_Out.Out_05_Sts.Out_SENSE/1
  in_DIAG_ACAN.BSG_EXPA.OUT_19_DIAG/1 -> out_OUT_FMSCAN.Tx_Out.Out_19_Sts.Out_DIAG/1
  in_IN_ACAN.BSG_EXPA.OUT_12_TD/1 -> out_OUT_FMSCAN.Tx_Out.Out_12_Sts.Out_TD/1, [boOut12TD]
  in_IN_ACAN.BSG_EXPA.OUT_09_HB_SENSE/1 -> out_OUT_FMSCAN.Tx_Out.Out_09_Sts.Out_SENSE/1
  in_DIAG_ACAN.BSG_EXPA.OUT_09_HB_DIAG/1 -> [Out09HBDiag], out_OUT_FMSCAN.Tx_Out.Out_09_Sts.Out_DIAG/1
  in_IN_ACAN.BSG_EXPA.OUT_19_SENSE/1 -> out_OUT_FMSCAN.Tx_Out.Out_19_Sts.Out_SENSE/1
  in_DIAG_ACAN.BSG_EXPA.OUT_24_DIAG/1 -> out_OUT_FMSCAN.Tx_Out.Out_24_Sts.Out_DIAG/1
  in_IN_ACAN.BSG_EXPA.OUT_01_HB_SENSE/1 -> out_OUT_FMSCAN.Tx_Out.Out_01_Sts.Out_SENSE/1
  in_DIAG_ACAN.BSG_EXPA.OUT_05_HB_DIAG/1 -> [Out05HBDiag], out_OUT_FMSCAN.Tx_Out.Out_05_Sts.Out_DIAG/1
  in_IN_ACAN.BSG_EXPA.OUT_26_SENSE/1 -> out_OUT_FMSCAN.Tx_Out.Out_26_Sts.Out_SENSE/1
  in_IN_ACAN.BSG_EXPA.OUT_08_HB_SENSE/1 -> out_OUT_FMSCAN.Tx_Out.Out_08_Sts.Out_SENSE/1
  in_IN_ACAN.BSG_EXPA.OUT_12_SENSE/1 -> out_OUT_FMSCAN.Tx_Out.Out_12_Sts.Out_SENSE/1
  in_IN_ACAN.BSG_EXPA.OUT_22_SENSE/1 -> out_OUT_FMSCAN.Tx_Out.Out_22_Sts.Out_SENSE/1
  in_DIAG_ACAN.BSG_EXPA.OUT_28_DIAG/1 -> out_OUT_FMSCAN.Tx_Out.Out_28_Sts.Out_DIAG/1
  in_DIAG_ACAN.BSG_EXPA.OUT_06_HB_DIAG/1 -> [Out06HBDiag], out_OUT_FMSCAN.Tx_Out.Out_06_Sts.Out_DIAG/1
  in_DIAG_ACAN.BSG_EXPA.OUT_03_DIAG/1 -> out_OUT_FMSCAN.Tx_Out.Out_03_Sts.Out_DIAG/1
  in_IN_ACAN.BSG_EXPA.OUT_10_HB_SENSE/1 -> out_OUT_FMSCAN.Tx_Out.Out_10_Sts.Out_SENSE/1
  in_IN_ACAN.BSG_EXPA.OUT_04_SENSE/1 -> out_OUT_FMSCAN.Tx_Out.Out_04_Sts.Out_SENSE/1
  in_DIAG_ACAN.BSG_EXPA.OUT_11_DIAG/1 -> out_OUT_FMSCAN.Tx_Out.Out_11_Sts.Out_DIAG/1
  in_DIAG_ACAN.BSG_EXPA.OUT_02_HB_DIAG/1 -> [Out02HBDiag], out_OUT_FMSCAN.Tx_Out.Out_02_Sts.Out_DIAG/1
  in_IN_ACAN.BSG_EXPA.OUT_21_SENSE/1 -> out_OUT_FMSCAN.Tx_Out.Out_21_Sts.Out_SENSE/1
  in_DIAG_ACAN.BSG_EXPA.OUT_01_HB_DIAG/1 -> [Out01HBDiag], out_OUT_FMSCAN.Tx_Out.Out_01_Sts.Out_DIAG/1
  in_IN_ACAN.BSG_EXPA.OUT_23_SENSE/1 -> out_OUT_FMSCAN.Tx_Out.Out_23_Sts.Out_SENSE/1
  Constant/1 -> out_OUT_FMSCAN.Rx_Ctrl.Out_Ctrl.MessageEnable/1, out_OUT_FMSCAN.Rx_Ctrl.Out_Mirror_HB_Ctrl.MessageEnable/1, out_OUT_FMSCAN.Rx_Ctrl.Out_HB_Ctrl.MessageEnable/1
  in_IN_FMSCAN.Rx_Ctrl.Out_Ctrl.MessageState/1 -> EQ/1(u1)
  Constant1/1 -> EQ/2(u2)
  EQ/1(y) -> [boCtrlMsgValid]
  [boCtrlMsgValid] -> AND13/1(u1), AND12/1(u1), AND17/1(u1), AND16/1(u1), AND15/1(u1), AND14/1(u1), AND11/1(u1), AND10/1(u1), AND9/1(u1), AND8/1(u1), AND7/1(u1), AND6/1(u1), AND5/1(u1), AND4/1(u1), AND3/1(u1), AND2/1(u1), AND1/1(u1), AND/1(u1)
  in_IN_FMSCAN.Rx_Ctrl.Out_Ctrl.Out_03_Ctrl/1 -> AND/2(u2)
  AND/1(y) -> Data Type Conversion12/1, out_OUT_ACAN.BSG_EXPA.OUT_03/1
  in_IN_FMSCAN.Rx_Ctrl.Out_Ctrl.Out_04_Ctrl/1 -> AND1/2(u2)
  AND1/1(y) -> Data Type Conversion13/1, out_OUT_ACAN.BSG_EXPA.OUT_04/1
  AND2/1(y) -> Data Type Conversion20/1, out_OUT_ACAN.BSG_EXPA.OUT_11/1
  AND3/1(y) -> Data Type Conversion21/1, out_OUT_ACAN.BSG_EXPA.OUT_13/1
  AND4/1(y) -> Data Type Conversion22/1, out_OUT_ACAN.BSG_EXPA.OUT_14/1
  AND5/1(y) -> Data Type Conversion23/1, out_OUT_ACAN.BSG_EXPA.OUT_15/1
  in_IN_FMSCAN.Rx_Ctrl.Out_Ctrl.Out_11_Ctrl/1 -> AND2/2(u2)
  in_IN_FMSCAN.Rx_Ctrl.Out_Ctrl.Out_13_Ctrl/1 -> AND3/2(u2)
  in_IN_FMSCAN.Rx_Ctrl.Out_Ctrl.Out_14_Ctrl/1 -> AND4/2(u2)
  in_IN_FMSCAN.Rx_Ctrl.Out_Ctrl.Out_15_Ctrl/1 -> AND5/2(u2)
  AND6/1(y) -> Data Type Conversion24/1, out_OUT_ACAN.BSG_EXPA.OUT_16/1
  AND7/1(y) -> Data Type Conversion25/1, out_OUT_ACAN.BSG_EXPA.OUT_17/1
  AND8/1(y) -> Data Type Conversion26/1, out_OUT_ACAN.BSG_EXPA.OUT_18/1
  AND9/1(y) -> Data Type Conversion27/1, out_OUT_ACAN.BSG_EXPA.OUT_19/1
  AND10/1(y) -> Data Type Conversion28/1, out_OUT_ACAN.BSG_EXPA.OUT_20/1
  AND11/1(y) -> Data Type Conversion29/1, out_OUT_ACAN.BSG_EXPA.OUT_22/1
  in_IN_FMSCAN.Rx_Ctrl.Out_Ctrl.Out_16_Ctrl/1 -> AND6/2(u2)
  in_IN_FMSCAN.Rx_Ctrl.Out_Ctrl.Out_17_Ctrl/1 -> AND7/2(u2)
  in_IN_FMSCAN.Rx_Ctrl.Out_Ctrl.Out_18_Ctrl/1 -> AND8/2(u2)
  in_IN_FMSCAN.Rx_Ctrl.Out_Ctrl.Out_19_Ctrl/1 -> AND9/2(u2)
  in_IN_FMSCAN.Rx_Ctrl.Out_Ctrl.Out_20_Ctrl/1 -> AND10/2(u2)
  in_IN_FMSCAN.Rx_Ctrl.Out_Ctrl.Out_22_Ctrl/1 -> AND11/2(u2)
  AND14/1(y) -> Data Type Conversion30/1, out_OUT_ACAN.BSG_EXPA.OUT_23/1
  AND15/1(y) -> Data Type Conversion31/1, out_OUT_ACAN.BSG_EXPA.OUT_24/1
  AND16/1(y) -> Data Type Conversion32/1, out_OUT_ACAN.BSG_EXPA.OUT_25/1
  AND17/1(y) -> Data Type Conversion33/1, out_OUT_ACAN.BSG_EXPA.OUT_26/1
  AND12/1(y) -> Data Type Conversion34/1, out_OUT_ACAN.BSG_EXPA.OUT_27/1
  AND13/1(y) -> Data Type Conversion35/1, out_OUT_ACAN.BSG_EXPA.OUT_28/1
  in_IN_FMSCAN.Rx_Ctrl.Out_Ctrl.Out_23_Ctrl/1 -> AND14/2(u2)
  in_IN_FMSCAN.Rx_Ctrl.Out_Ctrl.Out_24_Ctrl/1 -> AND15/2(u2)
  in_IN_FMSCAN.Rx_Ctrl.Out_Ctrl.Out_25_Ctrl/1 -> AND16/2(u2)
  in_IN_FMSCAN.Rx_Ctrl.Out_Ctrl.Out_26_Ctrl/1 -> AND17/2(u2)
  in_IN_FMSCAN.Rx_Ctrl.Out_Ctrl.Out_27_Ctrl/1 -> AND12/2(u2)
  in_IN_FMSCAN.Rx_Ctrl.Out_Ctrl.Out_28_Ctrl/1 -> AND13/2(u2)
  MOD_TrailerDetection_Ctrl_12/2 -> out_OUT_ACAN.BSG_EXPA.OUT_12_TD_START/1
  [boOut12TD] -> MOD_TrailerDetection_Ctrl_12/2
  [boOut12TDDiag] -> MOD_TrailerDetection_Ctrl_12/3
  Constant2/1 -> [u8TimeOut]
  [u8TimeOut] -> MOD_TrailerDetection_Ctrl_12/4
  [boCtrlMsgValid] -> AND18/1(u1)
  in_IN_FMSCAN.Rx_Ctrl.Out_Ctrl.Out_12_Ctrl/1 -> AND18/2(u2)
  AND18/1(y) -> [boOut12Rqst]
  MOD_TrailerDetection_Ctrl_12/1 -> [boOut12]
  [boOut12Rqst] -> MOD_TrailerDetection_Ctrl_12/1
  [boOut12] -> Data Type Conversion/1, out_OUT_ACAN.BSG_EXPA.OUT_12/1
  Data Type Conversion/1 -> out_OUT_FMSCAN.Tx_Out.Out_12_Sts.Out_STATUS/1
  [boOut21TDDiag] -> MOD_TrailerDetection_Ctrl_21/3
  MOD_TrailerDetection_Ctrl_21/2 -> out_OUT_ACAN.BSG_EXPA.OUT_21_TD_START/1
  in_IN_FMSCAN.Rx_Ctrl.Out_Ctrl.Out_21_Ctrl/1 -> AND19/2(u2)
  [boOut21] -> out_OUT_ACAN.BSG_EXPA.OUT_21/1, Data Type Conversion1/1
  [boOut21Rqst] -> MOD_TrailerDetection_Ctrl_21/1
  MOD_TrailerDetection_Ctrl_21/1 -> [boOut21]
  Data Type Conversion1/1 -> out_OUT_FMSCAN.Tx_Out.Out_21_Sts.Out_STATUS/1
  [u8TimeOut] -> MOD_TrailerDetection_Ctrl_21/4
  [boOut21TD] -> MOD_TrailerDetection_Ctrl_21/2
  [boCtrlMsgValid] -> AND19/1(u1)
  AND19/1(y) -> [boOut21Rqst]
  EQ1/1(y) -> [boHBCtrlMsgValid]
  in_IN_FMSCAN.Rx_Ctrl.Out_HB_Ctrl.MessageState/1 -> EQ1/1(u1)
  Constant3/1 -> EQ2/2(u2), EQ1/2(u2)
  [boHBCtrlMsgValid] -> Switch/2
  Data Type Conversion2/1 -> Switch/1
  in_IN_FMSCAN.Rx_Ctrl.Out_HB_Ctrl.Out_01_HB_Ctrl/1 -> Data Type Conversion2/1
  Constant4/1 -> Switch/3
  MOD_Hbridge_Ctrl12/1 -> Data Type Conversion10/1, out_OUT_ACAN.BSG_EXPA.OUT_01_HB/1
  in_IN_FMSCAN.Rx_Ctrl.Out_HB_Ctrl.Out_02_HB_Ctrl/1 -> Data Type Conversion3/1
  [boHBCtrlMsgValid] -> Switch1/2
  Constant5/1 -> Switch1/3
  Data Type Conversion3/1 -> Switch1/1
  MOD_Hbridge_Ctrl12/2 -> Data Type Conversion11/1, out_OUT_ACAN.BSG_EXPA.OUT_02_HB/1
  in_IN_FMSCAN.Rx_Ctrl.Out_HB_Ctrl.Out_05_HB_Ctrl/1 -> Data Type Conversion4/1
  MOD_Hbridge_Ctrl56/1 -> Data Type Conversion14/1, out_OUT_ACAN.BSG_EXPA.OUT_05_HB/1
  Constant6/1 -> Switch2/3
  [boHBCtrlMsgValid] -> Switch2/2
  Data Type Conversion4/1 -> Switch2/1
  in_IN_FMSCAN.Rx_Ctrl.Out_HB_Ctrl.Out_07_HB_Ctrl/1 -> Data Type Conversion6/1
  MOD_Hbridge_Ctrl78/1 -> Data Type Conversion16/1, out_OUT_ACAN.BSG_EXPA.OUT_07_HB/1
  [boHBCtrlMsgValid] -> Switch3/2
  Constant8/1 -> Switch4/3
  [boHBCtrlMsgValid] -> Switch4/2
  Data Type Conversion6/1 -> Switch4/1
  MOD_Hbridge_Ctrl56/2 -> Data Type Conversion15/1, out_OUT_ACAN.BSG_EXPA.OUT_06_HB/1
  Data Type Conversion7/1 -> Switch5/1
  MOD_Hbridge_Ctrl78/2 -> Data Type Conversion17/1, out_OUT_ACAN.BSG_EXPA.OUT_08_HB/1
  [boHBCtrlMsgValid] -> Switch5/2
  Constant9/1 -> Switch5/3
  Constant7/1 -> Switch3/3
  in_IN_FMSCAN.Rx_Ctrl.Out_HB_Ctrl.Out_06_HB_Ctrl/1 -> Data Type Conversion5/1
  Data Type Conversion5/1 -> Switch3/1
  in_IN_FMSCAN.Rx_Ctrl.Out_HB_Ctrl.Out_08_HB_Ctrl/1 -> Data Type Conversion7/1
  in_IN_FMSCAN.Rx_Ctrl.Out_HB_Ctrl.Out_10_HB_Ctrl/1 -> Data Type Conversion9/1
  MOD_Hbridge_Ctrl910/1 -> Data Type Conversion18/1, out_OUT_ACAN.BSG_EXPA.OUT_09_HB/1
  [boHBCtrlMsgValid] -> Switch7/2
  MOD_Hbridge_Ctrl910/2 -> Data Type Conversion19/1, out_OUT_ACAN.BSG_EXPA.OUT_10_HB/1
  Constant10/1 -> Switch6/3
  Data Type Conversion8/1 -> Switch6/1
  [boHBCtrlMsgValid] -> Switch6/2
  Constant11/1 -> Switch7/3
  in_IN_FMSCAN.Rx_Ctrl.Out_HB_Ctrl.Out_09_HB_Ctrl/1 -> Data Type Conversion8/1
  Data Type Conversion9/1 -> Switch7/1
  [boCtrlMsgValid] -> AND23/1(u1), AND22/1(u1), AND21/1(u1), AND20/1(u1)
  in_IN_FMSCAN.Rx_Ctrl.Out_Ctrl.Out_OLD_01_Ctrl/1 -> AND20/2(u2)
  MOD_Hbridge_Ctrl12/3 -> out_OUT_ACAN.BSG_EXPA.OUT_OLD_01/1
  in_IN_FMSCAN.Rx_Ctrl.Out_Ctrl.Out_OLD_02_Ctrl/1 -> AND21/2(u2)
  MOD_Hbridge_Ctrl56/3 -> out_OUT_ACAN.BSG_EXPA.OUT_OLD_03/1
  MOD_Hbridge_Ctrl910/3 -> out_OUT_ACAN.BSG_EXPA.OUT_OLD_04/1
  in_IN_FMSCAN.Rx_Ctrl.Out_Ctrl.Out_OLD_03_Ctrl/1 -> AND22/2(u2)
  in_IN_FMSCAN.Rx_Ctrl.Out_Ctrl.Out_OLD_04_Ctrl/1 -> AND23/2(u2)
  Data Type Conversion10/1 -> out_OUT_FMSCAN.Tx_Out.Out_01_Sts.Out_STATUS/1
  Data Type Conversion11/1 -> out_OUT_FMSCAN.Tx_Out.Out_02_Sts.Out_STATUS/1
  Data Type Conversion12/1 -> out_OUT_FMSCAN.Tx_Out.Out_03_Sts.Out_STATUS/1
  Data Type Conversion13/1 -> out_OUT_FMSCAN.Tx_Out.Out_04_Sts.Out_STATUS/1
  Data Type Conversion14/1 -> out_OUT_FMSCAN.Tx_Out.Out_05_Sts.Out_STATUS/1
  Data Type Conversion15/1 -> out_OUT_FMSCAN.Tx_Out.Out_06_Sts.Out_STATUS/1
  Data Type Conversion16/1 -> out_OUT_FMSCAN.Tx_Out.Out_07_Sts.Out_STATUS/1
  Data Type Conversion17/1 -> out_OUT_FMSCAN.Tx_Out.Out_08_Sts.Out_STATUS/1
  Data Type Conversion18/1 -> out_OUT_FMSCAN.Tx_Out.Out_09_Sts.Out_STATUS/1
  Data Type Conversion19/1 -> out_OUT_FMSCAN.Tx_Out.Out_10_Sts.Out_STATUS/1
  Data Type Conversion20/1 -> out_OUT_FMSCAN.Tx_Out.Out_11_Sts.Out_STATUS/1
  Data Type Conversion21/1 -> out_OUT_FMSCAN.Tx_Out.Out_13_Sts.Out_STATUS/1
  Data Type Conversion22/1 -> out_OUT_FMSCAN.Tx_Out.Out_14_Sts.Out_STATUS/1
  Data Type Conversion23/1 -> out_OUT_FMSCAN.Tx_Out.Out_15_Sts.Out_STATUS/1
  Data Type Conversion24/1 -> out_OUT_FMSCAN.Tx_Out.Out_16_Sts.Out_STATUS/1
  Data Type Conversion25/1 -> out_OUT_FMSCAN.Tx_Out.Out_17_Sts.Out_STATUS/1
  Data Type Conversion26/1 -> out_OUT_FMSCAN.Tx_Out.Out_18_Sts.Out_STATUS/1
  Data Type Conversion27/1 -> out_OUT_FMSCAN.Tx_Out.Out_19_Sts.Out_STATUS/1
  Data Type Conversion28/1 -> out_OUT_FMSCAN.Tx_Out.Out_20_Sts.Out_STATUS/1
  Data Type Conversion29/1 -> out_OUT_FMSCAN.Tx_Out.Out_22_Sts.Out_STATUS/1
  Data Type Conversion30/1 -> out_OUT_FMSCAN.Tx_Out.Out_23_Sts.Out_STATUS/1
  Data Type Conversion31/1 -> out_OUT_FMSCAN.Tx_Out.Out_24_Sts.Out_STATUS/1
  Data Type Conversion32/1 -> out_OUT_FMSCAN.Tx_Out.Out_25_Sts.Out_STATUS/1
  Data Type Conversion33/1 -> out_OUT_FMSCAN.Tx_Out.Out_26_Sts.Out_STATUS/1
  Data Type Conversion34/1 -> out_OUT_FMSCAN.Tx_Out.Out_27_Sts.Out_STATUS/1
  Data Type Conversion35/1 -> out_OUT_FMSCAN.Tx_Out.Out_28_Sts.Out_STATUS/1
  in_DIAG_ACAN.BSG_EXPA.OUT_29_HB_DIAG/1 -> out_OUT_FMSCAN.Tx_Out.Out_29_Sts.Out_DIAG/1
  in_DIAG_ACAN.BSG_EXPA.OUT_30_HB_DIAG/1 -> out_OUT_FMSCAN.Tx_Out.Out_30_Sts.Out_DIAG/1
  in_DIAG_ACAN.BSG_EXPA.OUT_31_HB_DIAG/1 -> out_OUT_FMSCAN.Tx_Out.Out_31_Sts.Out_DIAG/1
  in_DIAG_ACAN.BSG_EXPA.OUT_32_HB_DIAG/1 -> out_OUT_FMSCAN.Tx_Out.Out_32_Sts.Out_DIAG/1
  in_DIAG_ACAN.BSG_EXPA.OUT_33_HB_DIAG/1 -> out_OUT_FMSCAN.Tx_Out.Out_33_Sts.Out_DIAG/1
  in_DIAG_ACAN.BSG_EXPA.OUT_34_HB_DIAG/1 -> out_OUT_FMSCAN.Tx_Out.Out_34_Sts.Out_DIAG/1
  in_IN_FMSCAN.Rx_Ctrl.Out_Mirror_HB_Ctrl.MessageState/1 -> EQ2/1(u1)
  EQ2/1(y) -> [boHBMirrorCtrlMsgValid]
  Constant12/1 -> Switch8/3
  Switch8/1 -> out_OUT_ACAN.BSG_EXPA.OUT_29_HB/1, Data Type Conversion36/1
  Data Type Conversion36/1 -> out_OUT_FMSCAN.Tx_Out.Out_29_Sts.Out_STATUS/1
  Data Type Conversion37/1 -> Switch8/1
  in_IN_FMSCAN.Rx_Ctrl.Out_Mirror_HB_Ctrl.Out_29_HB_Ctrl/1 -> Data Type Conversion37/1
  [boHBMirrorCtrlMsgValid] -> Switch8/2
  Data Type Conversion38/1 -> out_OUT_FMSCAN.Tx_Out.Out_30_Sts.Out_STATUS/1
  in_IN_FMSCAN.Rx_Ctrl.Out_Mirror_HB_Ctrl.Out_30_HB_Ctrl/1 -> Data Type Conversion39/1
  [boHBMirrorCtrlMsgValid] -> Switch9/2
  Data Type Conversion39/1 -> Switch9/1
  Switch9/1 -> out_OUT_ACAN.BSG_EXPA.OUT_30_HB/1, Data Type Conversion38/1
  Constant13/1 -> Switch9/3
  Data Type Conversion40/1 -> out_OUT_FMSCAN.Tx_Out.Out_31_Sts.Out_STATUS/1
  in_IN_FMSCAN.Rx_Ctrl.Out_Mirror_HB_Ctrl.Out_31_HB_Ctrl/1 -> Data Type Conversion41/1
  [boHBMirrorCtrlMsgValid] -> Switch10/2
  Data Type Conversion41/1 -> Switch10/1
  Switch10/1 -> out_OUT_ACAN.BSG_EXPA.OUT_31_HB/1, Data Type Conversion40/1
  Constant14/1 -> Switch10/3
  Data Type Conversion42/1 -> out_OUT_FMSCAN.Tx_Out.Out_32_Sts.Out_STATUS/1
  in_IN_FMSCAN.Rx_Ctrl.Out_Mirror_HB_Ctrl.Out_32_HB_Ctrl/1 -> Data Type Conversion43/1
  [boHBMirrorCtrlMsgValid] -> Switch11/2
  Data Type Conversion43/1 -> Switch11/1
  Switch11/1 -> out_OUT_ACAN.BSG_EXPA.OUT_32_HB/1, Data Type Conversion42/1
  Constant15/1 -> Switch11/3
  Data Type Conversion44/1 -> out_OUT_FMSCAN.Tx_Out.Out_33_Sts.Out_STATUS/1
  in_IN_FMSCAN.Rx_Ctrl.Out_Mirror_HB_Ctrl.Out_33_HB_Ctrl/1 -> Data Type Conversion45/1
  [boHBMirrorCtrlMsgValid] -> Switch12/2
  Data Type Conversion45/1 -> Switch12/1
  Switch12/1 -> out_OUT_ACAN.BSG_EXPA.OUT_33_HB/1, Data Type Conversion44/1
  Constant16/1 -> Switch12/3
  Data Type Conversion46/1 -> out_OUT_FMSCAN.Tx_Out.Out_34_Sts.Out_STATUS/1
  in_IN_FMSCAN.Rx_Ctrl.Out_Mirror_HB_Ctrl.Out_34_HB_Ctrl/1 -> Data Type Conversion47/1
  [boHBMirrorCtrlMsgValid] -> Switch13/2
  Data Type Conversion47/1 -> Switch13/1
  Switch13/1 -> out_OUT_ACAN.BSG_EXPA.OUT_34_HB/1, Data Type Conversion46/1
  Constant17/1 -> Switch13/3
  in_IN_ACAN.BSG_EXPA.OUT_12_SENSE_PULSE/1 -> out_OUT_FMSCAN.Tx_Out.Out_12_TD_Sts.Out_SENSE_PULSE/1
  in_DIAG_ACAN.BSG_EXPA.OUT_12_SENSE_PULSE_DIAG/1 -> out_OUT_FMSCAN.Tx_Out.Out_12_TD_Sts.Out_SENSE_PULSE_DIAG/1
  in_IN_ACAN.BSG_EXPA.OUT_21_SENSE_PULSE/1 -> out_OUT_FMSCAN.Tx_Out.Out_21_TD_Sts.Out_SENSE_PULSE/1
  in_DIAG_ACAN.BSG_EXPA.OUT_21_SENSE_PULSE_DIAG/1 -> out_OUT_FMSCAN.Tx_Out.Out_21_TD_Sts.Out_SENSE_PULSE_DIAG/1
  [HMaxActivationTimeTime] -> MOD_Hbridge_Ctrl78/7
  [HOpenLoadDetectTime] -> MOD_Hbridge_Ctrl78/6
  [HBrakeTime] -> MOD_Hbridge_Ctrl78/5
  Switch4/1 -> MOD_Hbridge_Ctrl78/9
  Switch5/1 -> MOD_Hbridge_Ctrl78/10
  MOD_Hbridge_Ctrl78/3 -> out_OUT_ACAN.BSG_EXPA.OUT_OLD_02/1
  [Out07HBDiag] -> MOD_Hbridge_Ctrl78/3
  [Out08HBDiag] -> MOD_Hbridge_Ctrl78/4
  MOD_Hbridge_Ctrl78/4 -> Terminator3/1
  [InDig07] -> MOD_Hbridge_Ctrl78/1
  [InDig08] -> MOD_Hbridge_Ctrl78/2
  [HOpenLoadIntervalTime] -> MOD_Hbridge_Ctrl78/8
  [Out01HBDiag] -> MOD_Hbridge_Ctrl12/3
  [Out02HBDiag] -> MOD_Hbridge_Ctrl12/4
  [InDig01] -> MOD_Hbridge_Ctrl12/1
  [InDig02] -> MOD_Hbridge_Ctrl12/2
  [InDig05] -> MOD_Hbridge_Ctrl56/1
  [InDig06] -> MOD_Hbridge_Ctrl56/2
  [Out05HBDiag] -> MOD_Hbridge_Ctrl56/3
  [Out06HBDiag] -> MOD_Hbridge_Ctrl56/4
  in_IN_FMSCAN.Rx_Ctrl.Out_Ctrl.WorkingMode/1 -> AND24/1(u1)
  [WorkingMode] -> MOD_Hbridge_Ctrl78/12
  [WorkingMode] -> MOD_Hbridge_Ctrl910/12
  [HOpenLoadIntervalTime] -> MOD_Hbridge_Ctrl910/8
  [HBrakeTime] -> MOD_Hbridge_Ctrl910/5
  [HOpenLoadDetectTime] -> MOD_Hbridge_Ctrl910/6
  [HMaxActivationTimeTime] -> MOD_Hbridge_Ctrl910/7
  [InDig09] -> MOD_Hbridge_Ctrl910/1
  [Out09HBDiag] -> MOD_Hbridge_Ctrl910/3
  [InDig10] -> MOD_Hbridge_Ctrl910/2
  [Out10HBDiag] -> MOD_Hbridge_Ctrl910/4
  MOD_Hbridge_Ctrl910/4 -> Terminator1/1
  Switch6/1 -> MOD_Hbridge_Ctrl910/9
  Switch7/1 -> MOD_Hbridge_Ctrl910/10
  [OLD04] -> MOD_Hbridge_Ctrl910/11
  Switch/1 -> MOD_Hbridge_Ctrl12/9
  Switch1/1 -> MOD_Hbridge_Ctrl12/10
  [OLD01] -> MOD_Hbridge_Ctrl12/11
  MOD_Hbridge_Ctrl12/4 -> Terminator2/1
  [HMaxActivationTimeTime] -> MOD_Hbridge_Ctrl12/7
  [HBrakeTime] -> MOD_Hbridge_Ctrl12/5
  [HOpenLoadDetectTime] -> MOD_Hbridge_Ctrl12/6
  [HOpenLoadIntervalTime] -> MOD_Hbridge_Ctrl12/8
  [HOpenLoadIntervalTime] -> MOD_Hbridge_Ctrl56/8
  [HBrakeTime] -> MOD_Hbridge_Ctrl56/5
  [HOpenLoadDetectTime] -> MOD_Hbridge_Ctrl56/6
  [HMaxActivationTimeTime] -> MOD_Hbridge_Ctrl56/7
  Switch2/1 -> MOD_Hbridge_Ctrl56/9
  Switch3/1 -> MOD_Hbridge_Ctrl56/10
  [OLD03] -> MOD_Hbridge_Ctrl56/11
  [WorkingMode] -> MOD_Hbridge_Ctrl56/12
  MOD_Hbridge_Ctrl56/4 -> Terminator4/1
  [boCtrlMsgValid] -> AND24/2(u2)
  AND24/1(y) -> [WorkingMode]
  [OLD02] -> MOD_Hbridge_Ctrl78/11
  [WorkingMode] -> MOD_Hbridge_Ctrl12/12
  AND20/1(y) -> [OLD01]
  AND21/1(y) -> [OLD02]
  AND22/1(y) -> [OLD03]
  AND23/1(y) -> [OLD04]
  in_IN_NVM.Parameter.HBrakeTime/1 -> [HBrakeTime]
  in_IN_NVM.Parameter.HOpenLoadDetectTime/1 -> [HOpenLoadDetectTime]
  in_IN_NVM.Parameter.HMaxActivationTimeTime/1 -> [HMaxActivationTimeTime]
  in_IN_NVM.Parameter.HOpenLoadIntervalTime/1 -> [HOpenLoadIntervalTime]
